simulink model "Set_Speed"  (R2022b)
settings: configuration reference "CommonModelConfiguration" (kept outside this file)
(part 2 of 2)

== stateflow chart Set_Speed/SetSpeed ==
  state CARCONFIG_INVALID
    entry:
    PA_DSF_SetSpeed.Status = E_CommonStatus.NotPresent;
    PA_DSF_SetSpeed.Value = E_DSF_Value.DSF_Off;
    PA_DSF_SetSpeed.SetSpeed = 0;
    PA_DSF_SetSpeed.Offset = 0;
    SET_SetSpdSts = SetSpdSts1.SetSpdSts1_NoReq;
    SET_SetSpdForCrsCtrlFct = 0;
    SET_SetSpdForDispToDrvrVal = 0;
    settings: description=If carconfig isn't fulfilled, which says if there's a driver support function in the car, set the PA:s to the following values.
  state isError = errorCheck [function]
    (default) -> (junction 3420)
    (junction 3420) -> (junction 3421) [order 1] : [(GET_UsrSeldDrvrSpprtFct==DrvrSpprtFct.DrvrSpprtFct_ACC &&...
        | PA_DSF_Adaptive_Cruise_Control_Status==E_CommonStatus.SystemError) ||...
        | (GET_UsrSeldDrvrSpprtFct==DrvrSpprtFct.DrvrSpprtFct_CC &&...
        | PA_DSF_Cruise_Control_Status==E_CommonStatus.SystemError) ||...
        | (GET_UsrSeldDrvrSpprtFct==DrvrSpprtFct.DrvrSpprtFct_SL &&...
        | PA_DSF_Speed_Limiter_Status==E_CommonStatus.SystemError)]
    (junction 3420) -> (junction 3422) [order 2] : {isError = false;}
    (junction 3421) -> (junction 3423) : {isError = true;}
    (junction 3422) -> (junction 3423)
    (junction 3423) -> (junction 3424)
  state SYSTEM_OK
    state isActive = activationCheck [function]
      (default) -> (junction 3433)
      (junction 3433) -> (junction 3434) [order 1] : [(PA_DSF_Speed_Limiter_Status==E_CommonStatus.Available ||...
          | PA_DSF_Cruise_Control_Status==E_CommonStatus.Available ||...
          | PA_DSF_Adaptive_Cruise_Control_Status==E_CommonStatus.Available ||...
          | PA_SpeedControlFunction_Status==E_CommonStatus.Available) &&...
          | (GET_HmiAutnmsStsHmiAutnmsSts~=HmiAutnmsSts1.HmiAutnmsSts1_On ||...
          | cc_param_100~=3)]
      (junction 3433) -> (junction 3435) [order 2] : {isActive = 0;}
      (junction 3434) -> (junction 3436) : {isActive = 1;}
      (junction 3436) -> (junction 3435)
      (junction 3435) -> (junction 3437)
    state NOT_ACTIVE
      entry:
      PA_DSF_SetSpeed.Status = E_CommonStatus.Disabled;
      PA_DSF_SetSpeed.Value = E_DSF_Value.DSF_Off;
      PA_DSF_SetSpeed.SetSpeed = 0;
      PA_DSF_SetSpeed.Offset = 0;
      SET_SetSpdSts = SetSpdSts1.SetSpdSts1_NoReq;
      SET_SetSpdForCrsCtrlFct = 0;
      SET_SetSpdForDispToDrvrVal = 0;
      settings: description=No driver support function is available at the moment
    state ACTIVE
      entry:
      SET_SetSpdSts = SetSpdSts1.SetSpdSts1_NoReq;
      state ACTIVE_A2
        state MAX_AND_MIN_SETSPEED [parallel]
          %Sets the max and min set speed
          %the entry transition can be where ever, the correct value-
          %will be set the next step
          settings: executionOrder=1
          state retVal =MinSpeed(LCFG_SpeedMPH, LCFG_SpeedKPH) [function]
            (default) -> (junction 5350)
            (junction 5350) -> (junction 5351) [order 1] : [GET_SpdUnit==VehSpdIndcdUnit.VehSpdIndcdUnit_Kmph]
            (junction 5350) -> (junction 5352) [order 2] : {retVal=LCFG_SpeedMPH;}
            (junction 5351) -> (junction 5353) : {retVal=LCFG_SpeedKPH;}
            (junction 5353) -> (junction 5352)
            (junction 5352) -> (junction 5354)
            (junction 5354) -> (junction 5355) [order 1] : [retVal>CARCONFIG_MaxSetSpeed(cc_param_43)]
            (junction 5354) -> (junction 5356) [order 2]
            (junction 5355) -> (junction 5357) : {retVal=CARCONFIG_MaxSetSpeed(cc_param_43);}
            (junction 5357) -> (junction 5356)
            (junction 5356) -> (junction 5358)
          state retVal=Max_SetSpeed(LCFG_MPH, LCFG_KMPH) [function]
            (default) -> (junction 5374)
            (junction 5374) -> (junction 5375) [order 1] : [GET_SpdUnit==VehSpdIndcdUnit.VehSpdIndcdUnit_Mph]
            (junction 5374) -> (junction 5376) [order 2]
            (junction 5375) -> (junction 5378)
            (junction 5376) -> (junction 5377) [order 1] : [LCFG_KMPH>CARCONFIG_MaxSetSpeed(cc_param_43)]
            (junction 5378) -> (junction 5377) [order 1] : [LCFG_MPH>CARCONFIG_MaxSetSpeed(cc_param_43)]
            (junction 5376) -> (junction 5379) [order 2] : {retVal=LCFG_KMPH;}
            (junction 5377) -> (junction 5380) : {retVal=CARCONFIG_MaxSetSpeed(cc_param_43);}
            (junction 5378) -> (junction 5381) [order 2] : {retVal=LCFG_MPH;}
            (junction 5380) -> (junction 5379)
            (junction 5381) -> (junction 5380)
            (junction 5379) -> (junction 5382)
          state retval=CareKey(MaxSetSpeed) [function]
            (default) -> (junction 5401)
            (junction 5401) -> (junction 5402) [order 1] : [PA_VS_ReducedMaxSpeed_Status==E_CommonStatus.Available]
            (junction 5402) -> (junction 5403) [order 1] : [(GET_SpdUnit==VehSpdIndcdUnit.VehSpdIndcdUnit_Kmph &&...
                | SetSpeedMin<GET_KeyRstrictdActvSpeedLimit*(36/10)) ||...
                | (GET_SpdUnit==VehSpdIndcdUnit.VehSpdIndcdUnit_Mph &&...
                | SetSpeedMin<GET_KeyRstrictdActvSpeedLimit*(1152/512))]
            (junction 5401) -> (junction 5408) [order 2] : {retval=MaxSetSpeed}
            (junction 5402) -> (junction 5409) [order 2] : {retval=SetSpeedMin}
            (junction 5403) -> (junction 5405)
            (junction 5405) -> (junction 5404) [order 2] : [GET_SpdUnit==VehSpdIndcdUnit.VehSpdIndcdUnit_Kmph &&...
                | MaxSetSpeed>GET_KeyRstrictdActvSpeedLimit*(36/10)]
            (junction 5405) -> (junction 5406) [order 1] : [GET_SpdUnit==VehSpdIndcdUnit.VehSpdIndcdUnit_Mph &&...
                | MaxSetSpeed>GET_KeyRstrictdActvSpeedLimit*(1152/512)]
            (junction 5404) -> (junction 5407) : {retval=GET_KeyRstrictdActvSpeedLimit*(36/10)}
            (junction 5405) -> (junction 5410) [order 3] : {retval=MaxSetSpeed}
            (junction 5406) -> (junction 5411) : {retval=GET_KeyRstrictdActvSpeedLimit*(1152/512)}
            (junction 5407) -> (junction 5409)
            (junction 5410) -> (junction 5407)
            (junction 5411) -> (junction 5410)
            (junction 5409) -> (junction 5408)
            (junction 5408) -> (junction 5412)
          state CC
            entry, during: SetSpeedMin= MinSpeed(LCFG_CC_SetSpeedMinMPH, LCFG_CC_SetSpeedMinKPH);
            SetSpeedMax=CareKey(Max_SetSpeed(LCFG_CC_SetSpeedMaxMPH, LCFG_CC_SetSpeedMaxKPH));
          state SL
            entry, during: SetSpeedMin=MinSpeed(LCFG_SL_SetSpeedMinMPH, LCFG_SL_SetSpeedMinKPH);
            SetSpeedMax =CareKey( CARCONFIG_MaxSetSpeed(cc_param_43));
          state ACC
            entry, during: SetSpeedMin=MinSpeed(LCFG_SetSpeedMinMPH, LCFG_SetSpeedMinKPH);
            SetSpeedMax=CareKey(Max_SetSpeed(LCFG_SetSpeedMaxMPH, LCFG_SetSpeedMaxKPH));
          SYSTEM_OK.ACTIVE.ACTIVE_A2.MAX_AND_MIN_SETSPEED.ACC -> CC [order 1] : [PA_DSF_Cruise_Control_Status==E_CommonStatus.Available]
          CC -> SYSTEM_OK.ACTIVE.ACTIVE_A2.MAX_AND_MIN_SETSPEED.ACC [order 1] : [PA_DSF_Adaptive_Cruise_Control_Status==E_CommonStatus.Available]
          SYSTEM_OK.ACTIVE.ACTIVE_A2.MAX_AND_MIN_SETSPEED.SL -> CC [order 1] : [PA_DSF_Cruise_Control_Status==E_CommonStatus.Available]
          CC -> SYSTEM_OK.ACTIVE.ACTIVE_A2.MAX_AND_MIN_SETSPEED.SL [order 2] : [PA_DSF_Speed_Limiter_Status==E_CommonStatus.Available]
          (default) -> SYSTEM_OK.ACTIVE.ACTIVE_A2.MAX_AND_MIN_SETSPEED.ACC
          SYSTEM_OK.ACTIVE.ACTIVE_A2.MAX_AND_MIN_SETSPEED.SL -> SYSTEM_OK.ACTIVE.ACTIVE_A2.MAX_AND_MIN_SETSPEED.ACC [order 2] : [PA_DSF_Adaptive_Cruise_Control_Status==E_CommonStatus.Available]
          SYSTEM_OK.ACTIVE.ACTIVE_A2.MAX_AND_MIN_SETSPEED.ACC -> SYSTEM_OK.ACTIVE.ACTIVE_A2.MAX_AND_MIN_SETSPEED.SL [order 2] : [PA_DSF_Speed_Limiter_Status==E_CommonStatus.Available]
        state SETSPEED_HANDLING [parallel]
          entry: PA_DSF_SetSpeed.Status=E_CommonStatus.Available;
          PA_DSF_SetSpeed.Value=E_DSF_Value.DSF_Off;
          LCFG_Unit_Check();
          manualUpdate = false;
          during: unitChange();
          settings: executionOrder=2
          state SLA_UPDATE [parallel]
            during: Reset_Offset()
            settings: executionOrder=1
            state SETSPEED_REASON_RESET_COUNTER
            state SETSPEED_REASON_RESET
              entry: SET_SetSpdSts = SetSpdSts1.SetSpdSts1_NoReq;
            (default) -> SETSPEED_REASON_RESET
            SETSPEED_REASON_RESET -> SETSPEED_REASON_RESET_COUNTER : [slaUpdate()]
            SETSPEED_REASON_RESET_COUNTER -> SETSPEED_REASON_RESET [order 1] : [after(250, msec)]
            SETSPEED_REASON_RESET_COUNTER -> SETSPEED_REASON_RESET_COUNTER [order 2] : [slaUpdate()]
          state MANUAL_UPDATE [parallel]
            settings: executionOrder=2
            state OFF
              state STANDBY
                entry: PA_DSF_SetSpeed.Value=E_DSF_Value.DSF_Standby;
                manualUpdate = false;
            state ACTIVE
              entry,during: updateValue()
              state REQ_DISABLED
              state updateValue [function]
                (default) -> (junction 4911)
                (junction 4911) -> (junction 4910) [order 1] : [PA_DSF_Adaptive_Cruise_Control_Value == E_DSF_Value.DSF_StopMode]
                    |
                    | {PA_DSF_SetSpeed.Value = E_DSF_Value.DSF_Standby;}
                (junction 4910) -> (junction 4915)
                (junction 4911) -> (junction 4913) [order 2]
                (junction 4913) -> (junction 4912) [order 1] : [PA_DSF_SL_Warning_Value == E_OffOn.On ||...
                    | GET_AdjSpdLimnSts==AdjSpdLimnSts2.AdjSpdLimnSts2_Ovrd]
                    |
                    | {PA_DSF_SetSpeed.Value = E_DSF_Value.DSF_Overridden;}
                (junction 4912) -> (junction 4914)
                (junction 4913) -> (junction 4916) [order 2] : {PA_DSF_SetSpeed.Value = E_DSF_Value.DSF_Active;}
                (junction 4915) -> (junction 4914)
                (junction 4914) -> (junction 4916)
                (junction 4916) -> (junction 4917)
              state IDLE
                entry:
                manualUpdate = false;
                settings: description=In this state the application is waiting for steering wheel button events
              state SET_CURRENT_SPEED
                entry: PA_DSF_SetSpeed.SetSpeed = setCruiseSpeed(GET_VehSpdIndcdVal);
                SET_SetSpdSts = SetSpdSts1.SetSpdSts1_DrvrReq;
                manualUpdate = true;
              state SPEED_TAP
                entry: SET_SetSpdSts = SetSpdSts1.SetSpdSts1_DrvrReq;
                manualUpdate = true;
                settings: description="In this state the cruise speed is increased/decreased the amount specified by the Local Config parameter \"SetSpeedTap)"
                state retval=getIncrease(reqsetspeed) [function]
                  (default) -> (junction 4959) : {retval = setCruiseSpeed(reqsetspeed+ SetSpeedTap -...
                      | mod(reqsetspeed, SetSpeedTap));}
                state retval=getDecrease(reqsetspeed) [function]
                  (default) -> (junction 4964)
                  (junction 4964) -> (junction 4965) [order 1] : [mod(reqsetspeed, SetSpeedTap) > 0]
                  (junction 4964) -> (junction 4966) [order 2] : {retval = setCruiseSpeed(reqsetspeed - SetSpeedTap);}
                  (junction 4965) -> (junction 4967) : {retval = setCruiseSpeed(reqsetspeed -...
                      | mod(reqsetspeed, SetSpeedTap));}
                  (junction 4967) -> (junction 4966)
                  (junction 4966) -> (junction 4968)
                (default) -> (junction 4932)
                (junction 4932) -> (junction 4931) [order 1] : [INT_SWSInputData.Button == E_SWSButton.BtnL4Req]
                (junction 4931) -> (junction 4933)
                (junction 4932) -> (junction 4934) [order 2]
                (junction 4933) -> (junction 4936) [order 1] : [PA_DSF_Speed_Limit_Adaptation_Data~=0 && PA_DSF_Speed_Limit_Adaptation_Data<254 &&...
                    | PA_DSF_Speed_Limit_Adaptation_Value== E_DSF_Value.DSF_Active]
                (junction 4934) -> (junction 4935) [order 1] : [PA_DSF_Speed_Limit_Adaptation_Data~=0 && PA_DSF_Speed_Limit_Adaptation_Data<254 &&...
                    | PA_DSF_Speed_Limit_Adaptation_Value== E_DSF_Value.DSF_Active]
                (junction 4933) -> (junction 4937) [order 2] : {PA_DSF_SetSpeed.SetSpeed = getDecrease(PA_DSF_SetSpeed.SetSpeed);}
                (junction 4934) -> (junction 4938) [order 2] : {PA_DSF_SetSpeed.SetSpeed =getIncrease(PA_DSF_SetSpeed.SetSpeed);}
                (junction 4935) -> (junction 4939) : {PA_DSF_SetSpeed.Offset = setMaxSlOffset(getIncrease(setCruiseSpeed(SLA_Sign_Value)...
                    | + PA_DSF_SetSpeed.Offset) - setCruiseSpeed(SLA_Sign_Value));
                    | PA_DSF_SetSpeed.SetSpeed = setCruiseSpeed(SLA_Sign_Value)...
                    | + PA_DSF_SetSpeed.Offset;}
                (junction 4936) -> (junction 4940) : {PA_DSF_SetSpeed.Offset = setMaxSlOffset(getDecrease(setCruiseSpeed(SLA_Sign_Value)...
                    | + PA_DSF_SetSpeed.Offset) - setCruiseSpeed(SLA_Sign_Value));
                    | PA_DSF_SetSpeed.SetSpeed = setCruiseSpeed(SLA_Sign_Value) + PA_DSF_SetSpeed.Offset;}
                (junction 4940) -> (junction 4937)
                (junction 4937) -> (junction 4939)
                (junction 4939) -> (junction 4938)
                (junction 4938) -> (junction 4941)
              state SPEED_RAMP
                entry: fineTuningDone = false;
                SET_SetSpdSts = SetSpdSts1.SetSpdSts1_DrvrReq;
                manualUpdate = true;
                state ramp [function]
                  (default) -> (junction 4982)
                  (junction 4982) -> (junction 4983) [order 1] : [INT_SWSInputData.Button == E_SWSButton.BtnL4Req]
                  (junction 4982) -> (junction 4986) [order 2]
                  (junction 4983) -> (junction 4985)
                  (junction 4985) -> (junction 4984) [order 1] : [PA_DSF_Speed_Limit_Adaptation_Data~=0 && PA_DSF_Speed_Limit_Adaptation_Data<254 &&...
                      | (PA_DSF_Speed_Limit_Adaptation_Value== E_DSF_Value.DSF_Active)]
                  (junction 4984) -> (junction 4988) : {PA_DSF_SetSpeed.Offset = setMaxSlOffset(setCruiseSpeed(setCruiseSpeed(SLA_Sign_Value)...
                      | + PA_DSF_SetSpeed.Offset - SetSpeedRamp) - setCruiseSpeed(SLA_Sign_Value));
                      | PA_DSF_SetSpeed.SetSpeed = setCruiseSpeed(SLA_Sign_Value) + PA_DSF_SetSpeed.Offset;}
                  (junction 4985) -> (junction 4989) [order 2] : {PA_DSF_SetSpeed.SetSpeed = setCruiseSpeed(PA_DSF_SetSpeed.SetSpeed - SetSpeedRamp);}
                  (junction 4986) -> (junction 4987) [order 1] : [PA_DSF_Speed_Limit_Adaptation_Data~=0 && PA_DSF_Speed_Limit_Adaptation_Data<254 &&...
                      | PA_DSF_Speed_Limit_Adaptation_Value== E_DSF_Value.DSF_Active]
                  (junction 4987) -> (junction 4991) : {PA_DSF_SetSpeed.Offset = setMaxSlOffset(setCruiseSpeed(setCruiseSpeed(SLA_Sign_Value)...
                      | + PA_DSF_SetSpeed.Offset + SetSpeedRamp) - setCruiseSpeed(SLA_Sign_Value));
                      | PA_DSF_SetSpeed.SetSpeed = setCruiseSpeed(SLA_Sign_Value)...
                      | + PA_DSF_SetSpeed.Offset;}
                  (junction 4986) -> (junction 4990) [order 2] : {PA_DSF_SetSpeed.SetSpeed =setCruiseSpeed(PA_DSF_SetSpeed.SetSpeed+SetSpeedRamp);}
                  (junction 4988) -> (junction 4989)
                  (junction 4989) -> (junction 4991)
                  (junction 4991) -> (junction 4990)
                  (junction 4990) -> (junction 4992)
                state HOLD_SHORT
                  state IDLE
                  state RAMP
                    entry: ramp()
                  (default) -> SYSTEM_OK.ACTIVE.ACTIVE_A2.SETSPEED_HANDLING.MANUAL_UPDATE.ACTIVE.SPEED_RAMP.HOLD_SHORT.RAMP
                  SYSTEM_OK.ACTIVE.ACTIVE_A2.SETSPEED_HANDLING.MANUAL_UPDATE.ACTIVE.SPEED_RAMP.HOLD_SHORT.RAMP -> SYSTEM_OK.ACTIVE.ACTIVE_A2.SETSPEED_HANDLING.MANUAL_UPDATE.ACTIVE.SPEED_RAMP.HOLD_SHORT.IDLE
                  SYSTEM_OK.ACTIVE.ACTIVE_A2.SETSPEED_HANDLING.MANUAL_UPDATE.ACTIVE.SPEED_RAMP.HOLD_SHORT.IDLE -> SYSTEM_OK.ACTIVE.ACTIVE_A2.SETSPEED_HANDLING.MANUAL_UPDATE.ACTIVE.SPEED_RAMP.HOLD_SHORT.RAMP : after(LCFG_AdjustmentShort, sec)
                state HOLD_LONG_ADJUST_SPEED
                  state IDLE
                  state RAMP
                    entry: ramp()
                  (default) -> SYSTEM_OK.ACTIVE.ACTIVE_A2.SETSPEED_HANDLING.MANUAL_UPDATE.ACTIVE.SPEED_RAMP.HOLD_LONG_ADJUST_SPEED.IDLE
                  SYSTEM_OK.ACTIVE.ACTIVE_A2.SETSPEED_HANDLING.MANUAL_UPDATE.ACTIVE.SPEED_RAMP.HOLD_LONG_ADJUST_SPEED.RAMP -> SYSTEM_OK.ACTIVE.ACTIVE_A2.SETSPEED_HANDLING.MANUAL_UPDATE.ACTIVE.SPEED_RAMP.HOLD_LONG_ADJUST_SPEED.IDLE
                  SYSTEM_OK.ACTIVE.ACTIVE_A2.SETSPEED_HANDLING.MANUAL_UPDATE.ACTIVE.SPEED_RAMP.HOLD_LONG_ADJUST_SPEED.IDLE -> SYSTEM_OK.ACTIVE.ACTIVE_A2.SETSPEED_HANDLING.MANUAL_UPDATE.ACTIVE.SPEED_RAMP.HOLD_LONG_ADJUST_SPEED.RAMP : after(LCFG_AdjustmentLong, sec)
                state FINE_TUNING
                  state FINE_TUNING_DONE
                    entry: fineTuningDone = true
                  state No_RELEASE
                  state RAMP
                  (default) -> SYSTEM_OK.ACTIVE.ACTIVE_A2.SETSPEED_HANDLING.MANUAL_UPDATE.ACTIVE.SPEED_RAMP.FINE_TUNING.RAMP
                  SYSTEM_OK.ACTIVE.ACTIVE_A2.SETSPEED_HANDLING.MANUAL_UPDATE.ACTIVE.SPEED_RAMP.FINE_TUNING.RAMP -> SYSTEM_OK.ACTIVE.ACTIVE_A2.SETSPEED_HANDLING.MANUAL_UPDATE.ACTIVE.SPEED_RAMP.FINE_TUNING.No_RELEASE : [INT_SWSInputData.Event~=E_SWSEvent.Release]
                  SYSTEM_OK.ACTIVE.ACTIVE_A2.SETSPEED_HANDLING.MANUAL_UPDATE.ACTIVE.SPEED_RAMP.FINE_TUNING.No_RELEASE -> SYSTEM_OK.ACTIVE.ACTIVE_A2.SETSPEED_HANDLING.MANUAL_UPDATE.ACTIVE.SPEED_RAMP.FINE_TUNING.FINE_TUNING_DONE [order 2] : after(LCFG_FineTuning, sec)
                  (junction 5020) -> SYSTEM_OK.ACTIVE.ACTIVE_A2.SETSPEED_HANDLING.MANUAL_UPDATE.ACTIVE.SPEED_RAMP.FINE_TUNING.RAMP
                  SYSTEM_OK.ACTIVE.ACTIVE_A2.SETSPEED_HANDLING.MANUAL_UPDATE.ACTIVE.SPEED_RAMP.FINE_TUNING.No_RELEASE -> (junction 5021) [order 1] : [INT_SWSInputData.Event==E_SWSEvent.Release]
                  (junction 5021) -> (junction 5020) : {ramp()}
                (default) -> SYSTEM_OK.ACTIVE.ACTIVE_A2.SETSPEED_HANDLING.MANUAL_UPDATE.ACTIVE.SPEED_RAMP.HOLD_SHORT
                SYSTEM_OK.ACTIVE.ACTIVE_A2.SETSPEED_HANDLING.MANUAL_UPDATE.ACTIVE.SPEED_RAMP.HOLD_SHORT -> SYSTEM_OK.ACTIVE.ACTIVE_A2.SETSPEED_HANDLING.MANUAL_UPDATE.ACTIVE.SPEED_RAMP.HOLD_LONG_ADJUST_SPEED [order 1] : [INT_SWSInputData.Event == E_SWSEvent.HoldLong]
                SYSTEM_OK.ACTIVE.ACTIVE_A2.SETSPEED_HANDLING.MANUAL_UPDATE.ACTIVE.SPEED_RAMP.FINE_TUNING -> SYSTEM_OK.ACTIVE.ACTIVE_A2.SETSPEED_HANDLING.MANUAL_UPDATE.ACTIVE.SPEED_RAMP.HOLD_SHORT : [INT_SWSInputData.Event == E_SWSEvent.HoldShort]
                SYSTEM_OK.ACTIVE.ACTIVE_A2.SETSPEED_HANDLING.MANUAL_UPDATE.ACTIVE.SPEED_RAMP.HOLD_SHORT -> SYSTEM_OK.ACTIVE.ACTIVE_A2.SETSPEED_HANDLING.MANUAL_UPDATE.ACTIVE.SPEED_RAMP.FINE_TUNING [order 2] : [INT_SWSInputData.Event == E_SWSEvent.Release]
                SYSTEM_OK.ACTIVE.ACTIVE_A2.SETSPEED_HANDLING.MANUAL_UPDATE.ACTIVE.SPEED_RAMP.HOLD_LONG_ADJUST_SPEED -> SYSTEM_OK.ACTIVE.ACTIVE_A2.SETSPEED_HANDLING.MANUAL_UPDATE.ACTIVE.SPEED_RAMP.FINE_TUNING : [INT_SWSInputData.Event == E_SWSEvent.Release]
              (default) -> SYSTEM_OK.ACTIVE.ACTIVE_A2.SETSPEED_HANDLING.MANUAL_UPDATE.ACTIVE.REQ_DISABLED
              SYSTEM_OK.ACTIVE.ACTIVE_A2.SETSPEED_HANDLING.MANUAL_UPDATE.ACTIVE.IDLE -> SYSTEM_OK.ACTIVE.ACTIVE_A2.SETSPEED_HANDLING.MANUAL_UPDATE.ACTIVE.REQ_DISABLED [order 1] : [GET_AccSts==AccSts1.AccSts1_Stop ||...
                  | GET_AccSts==AccSts1.AccSts1_StopTmp]
              SYSTEM_OK.ACTIVE.ACTIVE_A2.SETSPEED_HANDLING.MANUAL_UPDATE.ACTIVE.REQ_DISABLED -> SYSTEM_OK.ACTIVE.ACTIVE_A2.SETSPEED_HANDLING.MANUAL_UPDATE.ACTIVE.IDLE : [INT_SWSInputData.Event == E_SWSEvent.Idle &&...
                  | GET_AccSts~=AccSts1.AccSts1_Stop &&...
                  | GET_AccSts~=AccSts1.AccSts1_StopTmp]
              SYSTEM_OK.ACTIVE.ACTIVE_A2.SETSPEED_HANDLING.MANUAL_UPDATE.ACTIVE.IDLE -> SYSTEM_OK.ACTIVE.ACTIVE_A2.SETSPEED_HANDLING.MANUAL_UPDATE.ACTIVE.SET_CURRENT_SPEED [order 2] : [(PA_DSF_Cruise_Control_Status==E_CommonStatus.Available ||...
                  | PA_DSF_Adaptive_Cruise_Control_Status==E_CommonStatus.Available) &&...
                  | GET_CrsCtrlOvrdn==OnOff1.OnOff1_On &&...
                  | INT_SWSInputData.Button == E_SWSButton.BtnL5Req &&...
                  | INT_SWSInputData.Event == E_SWSEvent.Push &&...
                  | GET_VehSpdIndcdVal>=PA_DSF_SetSpeed.SetSpeed]
              SYSTEM_OK.ACTIVE.ACTIVE_A2.SETSPEED_HANDLING.MANUAL_UPDATE.ACTIVE.SET_CURRENT_SPEED -> SYSTEM_OK.ACTIVE.ACTIVE_A2.SETSPEED_HANDLING.MANUAL_UPDATE.ACTIVE.IDLE : [INT_SWSInputData.Event == E_SWSEvent.Idle]
              SYSTEM_OK.ACTIVE.ACTIVE_A2.SETSPEED_HANDLING.MANUAL_UPDATE.ACTIVE.IDLE -> SYSTEM_OK.ACTIVE.ACTIVE_A2.SETSPEED_HANDLING.MANUAL_UPDATE.ACTIVE.SPEED_TAP [order 3] : [INT_SWSInputData.Event == E_SWSEvent.Release &&...
                  | (INT_SWSInputData.Button == E_SWSButton.BtnL4Req ||...
                  | INT_SWSInputData.Button == E_SWSButton.BtnL5Req)]
                settings: description=If the up or down button, from the left buttons group, is released.
              SYSTEM_OK.ACTIVE.ACTIVE_A2.SETSPEED_HANDLING.MANUAL_UPDATE.ACTIVE.SPEED_TAP -> SYSTEM_OK.ACTIVE.ACTIVE_A2.SETSPEED_HANDLING.MANUAL_UPDATE.ACTIVE.IDLE : [INT_SWSInputData.Event == E_SWSEvent.Idle]
              SYSTEM_OK.ACTIVE.ACTIVE_A2.SETSPEED_HANDLING.MANUAL_UPDATE.ACTIVE.IDLE -> SYSTEM_OK.ACTIVE.ACTIVE_A2.SETSPEED_HANDLING.MANUAL_UPDATE.ACTIVE.SPEED_RAMP [order 4] : [INT_SWSInputData.Event == E_SWSEvent.HoldShort &&...
                  | (INT_SWSInputData.Button == E_SWSButton.BtnL4Req ||...
                  | INT_SWSInputData.Button == E_SWSButton.BtnL5Req)]
              SYSTEM_OK.ACTIVE.ACTIVE_A2.SETSPEED_HANDLING.MANUAL_UPDATE.ACTIVE.SPEED_RAMP -> SYSTEM_OK.ACTIVE.ACTIVE_A2.SETSPEED_HANDLING.MANUAL_UPDATE.ACTIVE.IDLE : [INT_SWSInputData.Event == E_SWSEvent.Idle && fineTuningDone]
            (default) -> SYSTEM_OK.ACTIVE.ACTIVE_A2.SETSPEED_HANDLING.MANUAL_UPDATE.OFF
            SYSTEM_OK.ACTIVE.ACTIVE_A2.SETSPEED_HANDLING.MANUAL_UPDATE.ACTIVE -> STANDBY : [PA_DSF_Cruise_Control_Value==E_DSF_Value.DSF_Standby ||...
                | PA_DSF_Speed_Limiter_Value==E_DSF_Value.DSF_Standby ||...
                | PA_DSF_Adaptive_Cruise_Control_Value==E_DSF_Value.DSF_Standby]
            SYSTEM_OK.ACTIVE.ACTIVE_A2.SETSPEED_HANDLING.MANUAL_UPDATE.OFF -> SYSTEM_OK.ACTIVE.ACTIVE_A2.SETSPEED_HANDLING.MANUAL_UPDATE.ACTIVE [order 1] : [hasChangedTo(INT_CC_Event, E_DSF_Event.Activation) ||...
                | (PA_DSF_Cruise_Control_Value==E_DSF_Value.DSF_Active &&...
                | INT_CC_Event ==E_DSF_Event.NoReq) ||...
                | hasChangedTo(INT_SL_Event, E_DSF_Event.Activation) ||...
                | (PA_DSF_Speed_Limiter_Value==E_DSF_Value.DSF_Active &&...
                | INT_SL_Event ==E_DSF_Event.NoReq) ||...
                | hasChangedTo(INT_ACC_Event, E_DSF_Event.Activation) ||...
                | ((PA_DSF_Adaptive_Cruise_Control_Value==E_DSF_Value.DSF_Active ||...
                | PA_DSF_Adaptive_Cruise_Control_Value==E_DSF_Value.DSF_StopMode) &&...
                | INT_ACC_Event == E_DSF_Event.NoReq)]
                | {setDsfActivation()}
            SYSTEM_OK.ACTIVE.ACTIVE_A2.SETSPEED_HANDLING.MANUAL_UPDATE.OFF -> SYSTEM_OK.ACTIVE.ACTIVE_A2.SETSPEED_HANDLING.MANUAL_UPDATE.ACTIVE [order 2] : [hasChangedTo(INT_CC_Event, E_DSF_Event.Resume) ||...
                | hasChangedTo(INT_SL_Event, E_DSF_Event.Resume) ||...
                | hasChangedTo(INT_ACC_Event, E_DSF_Event.Resume)]
          state SLA_Speed_Change [function]
            state slaSetSpeedChange [function]
              (default) -> (junction 5076)
              (junction 5076) -> (junction 5077) [order 1] : [GET_SetSpdSelnForAutDrv==SetSpdSelnForAutDrv1.SetSpdSelnForAutDrv1_AdjSetSpdToCmngSpdLim]
              (junction 5076) -> (junction 5078) [order 2] : {SET_SetSpdSts = SetSpdSts1.SetSpdSts1_Lvl1;}
              (junction 5077) -> (junction 5079) : {SET_SetSpdSts = SetSpdSts1.SetSpdSts1_Lvl2;}
              (junction 5079) -> (junction 5078)
              (junction 5078) -> (junction 5080)
            (default) -> (junction 5040)
            (junction 5040) -> (junction 5039) [order 2]
            (junction 5040) -> (junction 5041) [order 1] : [PA_DSF_Adaptive_Cruise_Control_Status==E_CommonStatus.Available]
            (junction 5039) -> (junction 5043)
            (junction 5041) -> (junction 5044)
            (junction 5043) -> (junction 5042) [order 1] : [LCFG_SL_OffsetReset==false]
            (junction 5044) -> (junction 5045) [order 1] : [PA_DSF_Speed_Limit_Adaptation_Value~=E_DSF_Value.DSF_Standby]
            (junction 5043) -> (junction 5049) [order 2] : {PA_DSF_SetSpeed.SetSpeed=setCruiseSpeed(SLA_Sign_Value);
                | PA_DSF_SetSpeed.Offset=0;
                | SET_SetSpdSts = SetSpdSts1.SetSpdSts1_Lvl1;}
            (junction 5044) -> (junction 5051) [order 2] : {PA_DSF_SetSpeed.SetSpeed = setCruiseSpeed(GET_VehSpdIndcdVal - PA_DSF_SetSpeed.Offset);}
            (junction 5045) -> (junction 5046)
            (junction 5042) -> (junction 5048) : {PA_DSF_SetSpeed.Offset = setMaxSlOffset(setCruiseSpeed(setCruiseSpeed(SLA_Sign_Value)...
                | + PA_DSF_SetSpeed.Offset) - setCruiseSpeed(SLA_Sign_Value));
                | PA_DSF_SetSpeed.SetSpeed = setCruiseSpeed(SLA_Sign_Value)...
                | + PA_DSF_SetSpeed.Offset;
                | SET_SetSpdSts = SetSpdSts1.SetSpdSts1_Lvl1;}
            (junction 5046) -> (junction 5047) [order 1] : [PA_DSF_Speed_Limit_Adaptation_Data==254]
            (junction 5046) -> (junction 5052) [order 2] : {PA_DSF_SetSpeed.Offset = setCruiseSpeed(setCruiseSpeed(SLA_Sign_Value)...
                | + PA_DSF_SetSpeed.Offset) - setCruiseSpeed(SLA_Sign_Value);
                | PA_DSF_SetSpeed.SetSpeed = setCruiseSpeed(SLA_Sign_Value)...
                | + PA_DSF_SetSpeed.Offset;
                | slaSetSpeedChange()}
            (junction 5047) -> (junction 5053) : {PA_DSF_SetSpeed.Offset=0;
                | slaSetSpeedChange()}
            (junction 5048) -> (junction 5049)
            (junction 5049) -> (junction 5050)
            (junction 5051) -> (junction 5050)
            (junction 5052) -> (junction 5051)
            (junction 5053) -> (junction 5052)
            (junction 5050) -> (junction 5054)
          state retVal=slaUpdate [function]
            (default) -> (junction 5090)
            (junction 5090) -> (junction 5089) [order 1] : [hasChangedTo(PA_DSF_Speed_Limit_Adaptation_Value, E_DSF_Value.DSF_Standby)]
            (junction 5089) -> (junction 5098) : {retVal=false;
                | SLA_Speed_Change()}
            (junction 5090) -> (junction 5091) [order 2]
            (junction 5091) -> (junction 5092) [order 1] : [PA_DSF_Speed_Limit_Adaptation_Data~=0 &&...
                | PA_DSF_Speed_Limit_Adaptation_Data~=255]
            (junction 5091) -> (junction 5093) [order 2]
            (junction 5092) -> (junction 5094)
            (junction 5094) -> (junction 5095) [order 1] : [(PA_DSF_SetSpeed.SetSpeed~=0 &&...
                | hasChanged(PA_DSF_Speed_Limit_Adaptation_Data) &&...
                | (PA_DSF_Speed_Limit_Adaptation_Value==E_DSF_Value.DSF_Active ||...
                | PA_DSF_Speed_Limit_Adaptation_Value==E_DSF_Value.DSF_Selected)) ||...
                | hasChangedTo(PA_DSF_Speed_Limit_Adaptation_Value, E_DSF_Value.DSF_Active)]
            (junction 5094) -> (junction 5093) [order 2]
            (junction 5093) -> (junction 5096) : {retVal=false;}
            (junction 5095) -> (junction 5097) : {SLA_SpeedValue()
                | SLA_Speed_Change()
                | retVal=true}
            (junction 5097) -> (junction 5096)
            (junction 5098) -> (junction 5097)
            (junction 5096) -> (junction 5099)
            (junction 5099) -> (junction 5100) [order 1] : [manualUpdate==true]
            (junction 5099) -> (junction 5101) [order 2]
            (junction 5100) -> (junction 5102) : {retVal = true;}
            (junction 5102) -> (junction 5101)
            (junction 5101) -> (junction 5103)
          state SLA_SpeedValue [function]
            (default) -> (junction 5124) : {SLA_Sign_Value=PA_DSF_Speed_Limit_Adaptation_Data}
            (junction 5124) -> (junction 5125) [order 1] : [(GET_SpdLimUnit==SpdUnit1.SpdUnit1_KiloMtrPerHr &&...
                | GET_SpdUnit==VehSpdIndcdUnit.VehSpdIndcdUnit_Mph) ||...
                | (GET_SpdLimUnit==SpdUnit1.SpdUnit1_MilePerHr &&...
                | GET_SpdUnit==VehSpdIndcdUnit.VehSpdIndcdUnit_Kmph)]
            (junction 5124) -> (junction 5128) [order 2]
            (junction 5125) -> (junction 5126)
            (junction 5126) -> (junction 5127) [order 1] : [GET_SpdLimUnit==SpdUnit1.SpdUnit1_KiloMtrPerHr]
            (junction 5126) -> (junction 5129) [order 2] : {SLA_Sign_Value=103/64*SLA_Sign_Value;}
            (junction 5127) -> (junction 5130) : {SLA_Sign_Value=64/103*SLA_Sign_Value;}
            (junction 5129) -> (junction 5128) : {SLA_Sign_Value= floor(SLA_Sign_Value);}
                | %Round down to nearest integer
            (junction 5130) -> (junction 5129)
            (junction 5128) -> (junction 5131)
          state Reset_Offset [function]
            (default) -> (junction 5143)
            (junction 5143) -> (junction 5144) [order 1] : [PA_DSF_Speed_Limit_Adaptation_Value~= E_DSF_Value.DSF_Active &&...
                | PA_DSF_Speed_Limit_Adaptation_Value~= E_DSF_Value.DSF_Selected &&...
                | PA_DSF_Speed_Limit_Adaptation_Value~= E_DSF_Value.DSF_Standby]
            (junction 5144) -> (junction 5146) : {PA_DSF_SetSpeed.SetSpeed = PA_DSF_SetSpeed.SetSpeed...
                | - PA_DSF_SetSpeed.Offset;
                | PA_DSF_SetSpeed.Offset = 0;}
            (junction 5143) -> (junction 5145) [order 2]
            (junction 5146) -> (junction 5145)
            (junction 5145) -> (junction 5147)
          state retval=setMaxSlOffset(reqoffset) [function]
            state offset_max=LCFG_Offset [function]
              (default) -> (junction 5197)
              (junction 5197) -> (junction 5196) [order 1] : [GET_SpdUnit==VehSpdIndcdUnit.VehSpdIndcdUnit_Mph]
              (junction 5196) -> (junction 5198) : {offset_max=LCFG_SL_MaxOffsetMPH}
              (junction 5197) -> (junction 5199) [order 2] : {offset_max=LCFG_SL_MaxOffsetKPH}
              (junction 5198) -> (junction 5199)
              (junction 5199) -> (junction 5200)
            (default) -> (junction 5176)
            (junction 5176) -> (junction 5177) [order 1] : [PA_DSF_Speed_Limiter_Status==E_CommonStatus.Available &&...
                | abs(reqoffset)>LCFG_Offset()]
                | %absolute value of reqoffset is greater than LCFG_Offset
            (junction 5176) -> (junction 5180) [order 2] : {retval =reqoffset;}
            (junction 5177) -> (junction 5178)
            (junction 5178) -> (junction 5179) [order 1] : [(reqoffset)>0]
            (junction 5178) -> (junction 5181) [order 2] : {retval=-1*LCFG_Offset();}
            (junction 5179) -> (junction 5182) : {retval=LCFG_Offset();}
            (junction 5181) -> (junction 5180)
            (junction 5182) -> (junction 5181)
            (junction 5180) -> (junction 5183)
          state setDsfActivation [function]
            (default) -> (junction 5155)
            (junction 5155) -> (junction 5156) [order 1] : [SLA_Sign_Value~=0 && SLA_Sign_Value~=255 && (PA_DSF_Speed_Limit_Adaptation_Value== E_DSF_Value.DSF_Active ||...
                |  PA_DSF_Speed_Limit_Adaptation_Value== E_DSF_Value.DSF_Selected)]
            (junction 5155) -> (junction 5157) [order 2]
            (junction 5156) -> (junction 5161) : {PA_DSF_SetSpeed.SetSpeed = setCruiseSpeed(SLA_Sign_Value);
                | PA_DSF_SetSpeed.Offset=0;}
            (junction 5157) -> (junction 5158) [order 1] : [PA_DSF_Adaptive_Cruise_Control_Value==E_DSF_Value.DSF_StopMode]
            (junction 5157) -> (junction 5159) [order 2] : {PA_DSF_SetSpeed.SetSpeed = setCruiseSpeed(GET_VehSpdIndcdVal);}
            (junction 5158) -> (junction 5160) : {PA_DSF_SetSpeed.SetSpeed = setCruiseSpeed(SetSpeedMin);}
            (junction 5160) -> (junction 5159)
            (junction 5161) -> (junction 5160)
            (junction 5159) -> (junction 5162)
          state retval = setCruiseSpeed(val) [function]
            (default) -> (junction 5210)
            (junction 5210) -> (junction 5211)
            (junction 5211) -> (junction 5212) [order 1] : [val < SetSpeedMin]
            (junction 5212) -> (junction 5217) : {retval=SetSpeedMin;}
            (junction 5211) -> (junction 5213) [order 2]
            (junction 5213) -> (junction 5214) [order 1] : [val >SetSpeedMax]
            (junction 5213) -> (junction 5216) [order 2] : {retval=val;}
            (junction 5214) -> (junction 5215) : {retval=SetSpeedMax;}
            (junction 5217) -> (junction 5215)
            (junction 5215) -> (junction 5216)
            (junction 5216) -> (junction 5218)
          state LCFG_Unit_Check [function]
            (default) -> (junction 5231)
            (junction 5231) -> (junction 5232) [order 1] : [GET_SpdUnit==VehSpdIndcdUnit.VehSpdIndcdUnit_Mph]
            (junction 5231) -> (junction 5233) [order 2] : {SetSpeedTap=LCFG_SetSpeedTapKPH;
                | SetSpeedRamp=LCFG_SetSpeedRampKPH;
                | SetSpeedTap2=LCFG_SetSpeedTap2KPH;}
            (junction 5232) -> (junction 5234) : {SetSpeedTap=LCFG_SetSpeedTapMPH;
                | SetSpeedRamp=LCFG_SetSpeedRampMPH;
                | SetSpeedTap2=LCFG_SetSpeedTap2MPH;}
            (junction 5234) -> (junction 5233)
            (junction 5233) -> (junction 5235)
          state unitChange [function]
            (default) -> (junction 5243)
            (junction 5243) -> (junction 5244) [order 1] : [hasChanged(GET_SpdUnit)]
            (junction 5243) -> (junction 5247) [order 2]
            (junction 5244) -> (junction 5245) : {LCFG_Unit_Check();}
            (junction 5245) -> (junction 5246) [order 1] : [GET_SpdUnit==VehSpdIndcdUnit.VehSpdIndcdUnit_Mph]
            (junction 5245) -> (junction 5248) [order 2] : %Convert from MPH to KMPH while making sure we are within
                | % the allowed ranges
                | {PA_DSF_SetSpeed.SetSpeed = setCruiseSpeed(floor(103/64*PA_DSF_SetSpeed.SetSpeed));
                | PA_DSF_SetSpeed.Offset = setMaxSlOffset(floor(103/64*PA_DSF_SetSpeed.Offset));}
            (junction 5246) -> (junction 5249) : %Convert from KMPH to MPH while making sure we are within
                | % the allowed ranges
                | {PA_DSF_SetSpeed.SetSpeed = setCruiseSpeed(floor(64/103*PA_DSF_SetSpeed.SetSpeed));
                | PA_DSF_SetSpeed.Offset = setMaxSlOffset(floor(64/103*PA_DSF_SetSpeed.Offset));}
            (junction 5248) -> (junction 5247)
            (junction 5249) -> (junction 5248)
            (junction 5247) -> (junction 5250)
        state SETSPEED_OUTPUT [parallel]
          entry, during:
          SET_SetSpdForCrsCtrlFct=TrueVehicleSpeed(SetSpeedValue(PA_DSF_SetSpeed.SetSpeed, PA_SpeedControlFunction_Data, PA_SpeedControlFunction_Value));
          SET_SetSpdForDispToDrvrVal=PA_DSF_SetSpeed.SetSpeed;
          settings: executionOrder=3
          state ReqSpeed=SetSpeedValue(SetSpeed, SpeedControlData, SpeedControlValue) [function]
            (default) -> (junction 5267)
            (junction 5267) -> (junction 5268) [order 1] : [SpeedControlValue == E_OffOn.On]
            (junction 5267) -> (junction 5269) [order 2] : {ReqSpeed=SetSpeed;}
            (junction 5268) -> (junction 5270) : {ReqSpeed=SpeedControlData;}
            (junction 5270) -> (junction 5269)
            (junction 5269) -> (junction 5271)
          state ReqSpeed=TrueVehicleSpeed(SetSpeed) [function]
            state ConvertedSpeed = RevertConvertedSetSpeed(ConfigMid, ConfigTop, Speed, BreakpointMid, BreakpointTop) [function]
              (default) -> (junction 5306)
              (junction 5306) -> (junction 5307) [order 1] : [Speed==0]
              (junction 5307) -> (junction 5312) : {ConvertedSpeed=0;}
              (junction 5306) -> (junction 5308) [order 2]
              (junction 5308) -> (junction 5309) [order 1] : [Speed<=BreakpointMid]
              (junction 5308) -> (junction 5310) [order 2] : {ConvertedSpeed=Speed-(Speed-BreakpointMid)*(ConfigTop-ConfigMid)/(BreakpointTop-BreakpointMid)-ConfigMid;}
              (junction 5309) -> (junction 5311) : {ConvertedSpeed=Speed-(Speed*ConfigMid/BreakpointMid);}
              (junction 5311) -> (junction 5310)
              (junction 5312) -> (junction 5311)
              (junction 5310) -> (junction 5313)
            state OutPutSpeed =ConvertToMeterPerSecond (SpeedToConvert) [function]
              (default) -> (junction 5327)
              (junction 5327) -> (junction 5328) [order 1] : [GET_SpdUnit==VehSpdIndcdUnit.VehSpdIndcdUnit_Mph]
              (junction 5327) -> (junction 5329) [order 2] : {OutPutSpeed=SpeedToConvert*10/36;}
              (junction 5328) -> (junction 5330) : {OutPutSpeed=SpeedToConvert*515/1152;}
              (junction 5330) -> (junction 5329)
              (junction 5329) -> (junction 5331)
            (default) -> (junction 5282)
            (junction 5282) -> (junction 5281) [order 1] : [cc_param_160==1 || cc_param_160==3 || cc_param_160==5]
            (junction 5281) -> (junction 5287) : {ReqSpeed=ConvertToMeterPerSecond(SetSpeed);}
            (junction 5282) -> (junction 5283) [order 2]
            (junction 5283) -> (junction 5284) [order 1] : [GET_SpdUnit==VehSpdIndcdUnit.VehSpdIndcdUnit_Kmph]
            (junction 5283) -> (junction 5285) [order 2] : %Convert set speed to kph, remove offset and convert to m/s
                | {ReqSpeed = RevertConvertedSetSpeed(LCFG_AddedVehSpdMidOffset,...
                |  LCFG_AddedVehSpdTopOffset, SetSpeed*(103/64),...
                |  LCFG_AddedVehSpdMidOffset + LCFG_ActualVehSpdMid, ...
                |  LCFG_AddedVehSpdTopOffset + LCFG_ActualVehSpdTop)*10/36;}
            (junction 5284) -> (junction 5286) : %Remove offset and convert to m/s
                | {ReqSpeed = RevertConvertedSetSpeed(LCFG_AddedVehSpdMidOffset,...
                |  LCFG_AddedVehSpdTopOffset, SetSpeed,...
                |  LCFG_AddedVehSpdMidOffset + LCFG_ActualVehSpdMid,...
                |  LCFG_AddedVehSpdTopOffset + LCFG_ActualVehSpdTop)*10/36;}
            (junction 5286) -> (junction 5285)
            (junction 5287) -> (junction 5286)
            (junction 5285) -> (junction 5288)
      state ACTIVE_A3
        entry:
        PA_DSF_SetSpeed.Status = E_CommonStatus.Disabled;
        PA_DSF_SetSpeed.Value = E_DSF_Value.DSF_Off;
        PA_DSF_SetSpeed.SetSpeed = 0;
        PA_DSF_SetSpeed.Offset = 0;
        SET_SetSpdSts = SetSpdSts1.SetSpdSts1_NoReq;
        SET_SetSpdForCrsCtrlFct = 0;
        SET_SetSpdForDispToDrvrVal = 0;
        state MAX_AND_MIN_SETSPEED [parallel]
          %Sets the max and min set speed,
          %the entry transition can be wherever,
          %the correct value will be set the next step
          settings: executionOrder=1
          state retVal = Min_SetSpeed(MinSpeedMPH, MinSpeedKPH) [function]
            (default) -> (junction 4424)
            (junction 4424) -> (junction 4425) [order 1] : [GET_SpdUnit==VehSpdIndcdUnit.VehSpdIndcdUnit_Kmph]
            (junction 4424) -> (junction 4426) [order 2] : {retVal = MinSpeedMPH;}
            (junction 4425) -> (junction 4427) : {retVal = MinSpeedKPH;}
            (junction 4427) -> (junction 4426)
            (junction 4426) -> (junction 4428)
            (junction 4428) -> (junction 4429) [order 1] : [retVal>CARCONFIG_MaxSetSpeed(cc_param_43)]
            (junction 4428) -> (junction 4430) [order 2]
            (junction 4429) -> (junction 4431) : {retVal = CARCONFIG_MaxSetSpeed(cc_param_43);}
            (junction 4431) -> (junction 4430)
            (junction 4430) -> (junction 4432)
          state retVal = Max_SetSpeed(MaxSpeedMPH, MaxSpeedKPH) [function]
            (default) -> (junction 4451)
            (junction 4451) -> (junction 4452) [order 1] : [GET_SpdUnit==VehSpdIndcdUnit.VehSpdIndcdUnit_Mph]
            (junction 4451) -> (junction 4453) [order 2]
            (junction 4452) -> (junction 4455)
            (junction 4453) -> (junction 4454) [order 1] : [MaxSpeedKPH>CARCONFIG_MaxSetSpeed(cc_param_43)]
            (junction 4455) -> (junction 4454) [order 1] : [MaxSpeedMPH>CARCONFIG_MaxSetSpeed(cc_param_43)]
            (junction 4453) -> (junction 4456) [order 2] : {retVal = MaxSpeedKPH;}
            (junction 4454) -> (junction 4457) : {retVal = CARCONFIG_MaxSetSpeed(cc_param_43);}
            (junction 4455) -> (junction 4458) [order 2] : {retVal = MaxSpeedMPH;}
            (junction 4457) -> (junction 4456)
            (junction 4458) -> (junction 4457)
            (junction 4456) -> (junction 4459)
          state retval = CareKey(MaxSetSpeed) [function]
            (default) -> (junction 4475)
            (junction 4475) -> (junction 4476) [order 1] : [PA_VS_ReducedMaxSpeed_Status==...
                | E_CommonStatus.Available]
            (junction 4476) -> (junction 4477) [order 1] : [(GET_SpdUnit==VehSpdIndcdUnit.VehSpdIndcdUnit_Kmph &&...
                | SetSpeedMin<GET_KeyRstrictdActvSpeedLimit*(36/10)) ||...
                | (GET_SpdUnit==VehSpdIndcdUnit.VehSpdIndcdUnit_Mph &&...
                | SetSpeedMin<GET_KeyRstrictdActvSpeedLimit*(1152/512))]
            (junction 4475) -> (junction 4482) [order 2] : {retval = MaxSetSpeed;}
            (junction 4476) -> (junction 4483) [order 2] : {retval = SetSpeedMin;}
            (junction 4477) -> (junction 4479)
            (junction 4479) -> (junction 4478) [order 2] : [GET_SpdUnit==VehSpdIndcdUnit.VehSpdIndcdUnit_Kmph &&...
                | MaxSetSpeed>GET_KeyRstrictdActvSpeedLimit*(36/10)]
            (junction 4479) -> (junction 4480) [order 1] : [GET_SpdUnit==VehSpdIndcdUnit.VehSpdIndcdUnit_Mph &&...
                | MaxSetSpeed>GET_KeyRstrictdActvSpeedLimit*(1152/512)]
            (junction 4478) -> (junction 4481) : {retval = GET_KeyRstrictdActvSpeedLimit*(36/10);}
            (junction 4479) -> (junction 4484) [order 3] : {retval = MaxSetSpeed;}
            (junction 4480) -> (junction 4485) : {retval = GET_KeyRstrictdActvSpeedLimit*(1152/512);}
            (junction 4483) -> (junction 4482)
            (junction 4481) -> (junction 4483)
            (junction 4484) -> (junction 4481)
            (junction 4485) -> (junction 4484)
            (junction 4482) -> (junction 4486)
          state ACC
            entry, during:
            SetSpeedMin =...
            Min_SetSpeed(LCFG_SetSpeedMinMPH_A3, LCFG_SetSpeedMinKPH_A3);
            SetSpeedMax =...
            CareKey(Max_SetSpeed(LCFG_SetSpeedMaxMPH, LCFG_SetSpeedMaxKPH));
          state SL
            entry, during:
            SetSpeedMin =...
            Min_SetSpeed(LCFG_SetSpeedMinMPH_A3, LCFG_SetSpeedMinKPH_A3);
            SetSpeedMax =...
            CareKey(CARCONFIG_MaxSetSpeed(cc_param_43));
          (default) -> SYSTEM_OK.ACTIVE.ACTIVE_A3.MAX_AND_MIN_SETSPEED.ACC
          SYSTEM_OK.ACTIVE.ACTIVE_A3.MAX_AND_MIN_SETSPEED.SL -> SYSTEM_OK.ACTIVE.ACTIVE_A3.MAX_AND_MIN_SETSPEED.ACC : %ACC selected
              | [PA_DSF_Adaptive_Cruise_Control_Status==E_CommonStatus.Available]
          SYSTEM_OK.ACTIVE.ACTIVE_A3.MAX_AND_MIN_SETSPEED.ACC -> SYSTEM_OK.ACTIVE.ACTIVE_A3.MAX_AND_MIN_SETSPEED.SL : %SL selected
              | [PA_DSF_Speed_Limiter_Status==E_CommonStatus.Available]
        state SETSPEED_HANDLING [parallel]
          entry:
          PA_DSF_SetSpeed.Status = E_CommonStatus.Available;
          PA_DSF_SetSpeed.Value = E_DSF_Value.DSF_Off;
          LCFG_Unit_Check();
          during:
          unitChange();
          settings: executionOrder=2
          state MANUAL_UPDATE [parallel]
            settings: executionOrder=1
            state OFF
              entry:
              PA_DSF_SetSpeed.Value =...
              E_DSF_Value.DSF_Standby;
            state ACTIVE
              entry,during: updateValue()
              state REQ_DISABLED
              state updateValue [function]
                (default) -> (junction 4526)
                (junction 4526) -> (junction 4527) [order 1] : [PA_DSF_Adaptive_Cruise_Control_Value==E_DSF_Value.DSF_StopMode]
                    | {PA_DSF_SetSpeed.Value = E_DSF_Value.DSF_Standby;}
                (junction 4526) -> (junction 4528) [order 2]
                (junction 4527) -> (junction 4531)
                (junction 4528) -> (junction 4529) [order 1] : [GET_CrsCtrlOvrdn==OnOff1.OnOff1_On ||...
                    | PA_DSF_SL_Warning_Value==E_OffOn.On ||...
                    | GET_AdjSpdLimnSts==AdjSpdLimnSts2.AdjSpdLimnSts2_Ovrd]
                    | {PA_DSF_SetSpeed.Value = E_DSF_Value.DSF_Overridden;}
                (junction 4529) -> (junction 4530)
                (junction 4528) -> (junction 4532) [order 2] : {PA_DSF_SetSpeed.Value = E_DSF_Value.DSF_Active;}
                (junction 4531) -> (junction 4530)
                (junction 4530) -> (junction 4532)
                (junction 4532) -> (junction 4533)
              state retval = validSLA [function]
                (default) -> (junction 4546) : {retval = PA_DSF_Speed_Limit_Adaptation_Data~=0 &&...
                    | PA_DSF_Speed_Limit_Adaptation_Data<254 &&...
                    | (PA_DSF_Speed_Limit_Adaptation_Value==E_DSF_Value.DSF_Active ||...
                    | PA_DSF_Speed_Limit_Adaptation_Value==E_DSF_Value.DSF_Standby);}
              state offset_max = limitOffset [function]
                (default) -> (junction 4550)
                (junction 4550) -> (junction 4551) [order 1] : [GET_SpdUnit==VehSpdIndcdUnit.VehSpdIndcdUnit_Mph]
                (junction 4550) -> (junction 4552) [order 2] : {offset_max = LCFG_SL_MaxOffsetKPH;}
                (junction 4551) -> (junction 4553) : {offset_max = LCFG_SL_MaxOffsetMPH;}
                (junction 4553) -> (junction 4552)
                (junction 4552) -> (junction 4554)
              state IDLE
                settings: description=In this state the application is waiting for steering wheel button events
              state SET_CURRENT_SPEED
                entry:
                PA_DSF_SetSpeed.SetSpeed = limitCruiseSpeed(GET_VehSpdIndcdVal);
                SET_SetSpdForDispToDrvrVal = PA_DSF_SetSpeed.SetSpeed;
                SetSpeedControlOutput(PA_DSF_SetSpeed.SetSpeed)
              state SPEED_TAP
                settings: description="In this state the cruise speed is increased/decreased the amount specified by the Local Config parameter \"SetSpeedTap)"
                state retval = getIncrease(reqsetspeed) [function]
                  (default) -> (junction 4592) : {retval = limitCruiseSpeed(reqsetspeed + SetSpeedTap -...
                      | mod(reqsetspeed, SetSpeedTap));}
                state retval = getDecrease(reqsetspeed) [function]
                  (default) -> (junction 4597)
                  (junction 4597) -> (junction 4598) [order 1] : [mod(reqsetspeed, SetSpeedTap) > 0]
                  (junction 4597) -> (junction 4599) [order 2] : {retval = limitCruiseSpeed(reqsetspeed - SetSpeedTap);}
                  (junction 4598) -> (junction 4600) : {retval = limitCruiseSpeed(reqsetspeed -...
                      | mod(reqsetspeed, SetSpeedTap));}
                  (junction 4600) -> (junction 4599)
                  (junction 4599) -> (junction 4601)
                (default) -> (junction 4564)
                (junction 4564) -> (junction 4565) [order 1] : %Set speed decrease (down button)
                    | [INT_SWSInputData.Button == E_SWSButton.BtnL4Req]
                (junction 4564) -> (junction 4566) [order 2] : %Set speed increase
                    | {PA_DSF_SetSpeed.SetSpeed = getIncrease(PA_DSF_SetSpeed.SetSpeed);}
                (junction 4565) -> (junction 4568) : %Set speed decrease
                    | {PA_DSF_SetSpeed.SetSpeed = getDecrease(PA_DSF_SetSpeed.SetSpeed);}
                (junction 4566) -> (junction 4567) [order 1] : %SLA valid, SL active and max offset exceeded
                    | [validSLA && PA_DSF_Speed_Limiter_Status==E_CommonStatus.Available &&...
                    | PA_DSF_SetSpeed.SetSpeed - limitCruiseSpeed(SLA_Sign_Value) > limitOffset]
                (junction 4568) -> (junction 4569) [order 1] : %SLA valid, SL active and max offset exceeded
                    | [validSLA && PA_DSF_Speed_Limiter_Status==E_CommonStatus.Available &&...
                    | PA_DSF_SetSpeed.SetSpeed - limitCruiseSpeed(SLA_Sign_Value) < -limitOffset]
                (junction 4566) -> (junction 4570) [order 2]
                (junction 4568) -> (junction 4572) [order 2]
                (junction 4567) -> (junction 4571) : %Limit to max offset from current speed limit
                    | {PA_DSF_SetSpeed.SetSpeed =...
                    | limitCruiseSpeed(SLA_Sign_Value) + limitOffset;}
                (junction 4569) -> (junction 4573) : %Limit to max offset from current speed limit
                    | {PA_DSF_SetSpeed.SetSpeed =...
                    | limitCruiseSpeed(SLA_Sign_Value) - limitOffset;}
                (junction 4571) -> (junction 4570)
                (junction 4572) -> (junction 4571)
                (junction 4573) -> (junction 4572)
                (junction 4570) -> (junction 4574) : %Set new output speed values for display and control
                    | {SET_SetSpdForDispToDrvrVal = PA_DSF_SetSpeed.SetSpeed;
                    | SetSpeedControlOutput(PA_DSF_SetSpeed.SetSpeed)}
              state SPEED_RAMP
                entry:
                fineTuningDone = false;
                state ramp [function]
                  (default) -> (junction 4615)
                  (junction 4615) -> (junction 4616) [order 1] : %Set speed decrease (down button)
                      | [INT_SWSInputData.Button==E_SWSButton.BtnL4Req]
                  (junction 4615) -> (junction 4617) [order 2] : %Increase set speed
                      | {PA_DSF_SetSpeed.SetSpeed =...
                      | limitCruiseSpeed(PA_DSF_SetSpeed.SetSpeed + SetSpeedRamp);}
                  (junction 4616) -> (junction 4619) : %Decrease set speed
                      | {PA_DSF_SetSpeed.SetSpeed =...
                      | limitCruiseSpeed(PA_DSF_SetSpeed.SetSpeed - SetSpeedRamp);}
                  (junction 4617) -> (junction 4618) [order 1] : %SLA valid, SL active and max offset exceeded
                      | [validSLA && PA_DSF_Speed_Limiter_Status==E_CommonStatus.Available &&...
                      | PA_DSF_SetSpeed.SetSpeed - limitCruiseSpeed(SLA_Sign_Value) > limitOffset]
                  (junction 4619) -> (junction 4620) [order 1] : %SLA valid, SL active and max offset exceeded
                      | [validSLA && PA_DSF_Speed_Limiter_Status==E_CommonStatus.Available &&...
                      | PA_DSF_SetSpeed.SetSpeed - limitCruiseSpeed(SLA_Sign_Value) < -limitOffset]
                  (junction 4618) -> (junction 4622) : %Limit to max offset from current speed limit
                      | {PA_DSF_SetSpeed.SetSpeed =...
                      | limitCruiseSpeed(SLA_Sign_Value) + limitOffset;}
                  (junction 4620) -> (junction 4624) : %Limit to max offset from current speed limit
                      | {PA_DSF_SetSpeed.SetSpeed =...
                      | limitCruiseSpeed(SLA_Sign_Value) - limitOffset;}
                  (junction 4617) -> (junction 4621) [order 2]
                  (junction 4619) -> (junction 4623) [order 2]
                  (junction 4622) -> (junction 4621)
                  (junction 4623) -> (junction 4622)
                  (junction 4624) -> (junction 4623)
                  (junction 4621) -> (junction 4625) : %Set new output speed values for display and control
                      | {SET_SetSpdForDispToDrvrVal = PA_DSF_SetSpeed.SetSpeed;
                      | SetSpeedControlOutput(PA_DSF_SetSpeed.SetSpeed)}
                state HOLD_SHORT
                  state RAMP
                    entry: ramp()
                  state IDLE
                  (default) -> SYSTEM_OK.ACTIVE.ACTIVE_A3.SETSPEED_HANDLING.MANUAL_UPDATE.ACTIVE.SPEED_RAMP.HOLD_SHORT.RAMP
                  SYSTEM_OK.ACTIVE.ACTIVE_A3.SETSPEED_HANDLING.MANUAL_UPDATE.ACTIVE.SPEED_RAMP.HOLD_SHORT.RAMP -> SYSTEM_OK.ACTIVE.ACTIVE_A3.SETSPEED_HANDLING.MANUAL_UPDATE.ACTIVE.SPEED_RAMP.HOLD_SHORT.IDLE
                  SYSTEM_OK.ACTIVE.ACTIVE_A3.SETSPEED_HANDLING.MANUAL_UPDATE.ACTIVE.SPEED_RAMP.HOLD_SHORT.IDLE -> SYSTEM_OK.ACTIVE.ACTIVE_A3.SETSPEED_HANDLING.MANUAL_UPDATE.ACTIVE.SPEED_RAMP.HOLD_SHORT.RAMP : after(LCFG_AdjustmentShort, sec)
                state HOLD_LONG_ADJUST_SPEED
                  state IDLE
                  state RAMP
                    entry: ramp()
                  (default) -> SYSTEM_OK.ACTIVE.ACTIVE_A3.SETSPEED_HANDLING.MANUAL_UPDATE.ACTIVE.SPEED_RAMP.HOLD_LONG_ADJUST_SPEED.IDLE
                  SYSTEM_OK.ACTIVE.ACTIVE_A3.SETSPEED_HANDLING.MANUAL_UPDATE.ACTIVE.SPEED_RAMP.HOLD_LONG_ADJUST_SPEED.IDLE -> SYSTEM_OK.ACTIVE.ACTIVE_A3.SETSPEED_HANDLING.MANUAL_UPDATE.ACTIVE.SPEED_RAMP.HOLD_LONG_ADJUST_SPEED.RAMP : after(LCFG_AdjustmentLong, sec)
                  SYSTEM_OK.ACTIVE.ACTIVE_A3.SETSPEED_HANDLING.MANUAL_UPDATE.ACTIVE.SPEED_RAMP.HOLD_LONG_ADJUST_SPEED.RAMP -> SYSTEM_OK.ACTIVE.ACTIVE_A3.SETSPEED_HANDLING.MANUAL_UPDATE.ACTIVE.SPEED_RAMP.HOLD_LONG_ADJUST_SPEED.IDLE
                state FINE_TUNING
                  state FINE_TUNING_DONE
                    entry: fineTuningDone = true
                  state No_RELEASE
                  state RAMP
                  (default) -> SYSTEM_OK.ACTIVE.ACTIVE_A3.SETSPEED_HANDLING.MANUAL_UPDATE.ACTIVE.SPEED_RAMP.FINE_TUNING.RAMP
                  SYSTEM_OK.ACTIVE.ACTIVE_A3.SETSPEED_HANDLING.MANUAL_UPDATE.ACTIVE.SPEED_RAMP.FINE_TUNING.RAMP -> SYSTEM_OK.ACTIVE.ACTIVE_A3.SETSPEED_HANDLING.MANUAL_UPDATE.ACTIVE.SPEED_RAMP.FINE_TUNING.No_RELEASE : [INT_SWSInputData.Event~=E_SWSEvent.Release]
                  SYSTEM_OK.ACTIVE.ACTIVE_A3.SETSPEED_HANDLING.MANUAL_UPDATE.ACTIVE.SPEED_RAMP.FINE_TUNING.No_RELEASE -> SYSTEM_OK.ACTIVE.ACTIVE_A3.SETSPEED_HANDLING.MANUAL_UPDATE.ACTIVE.SPEED_RAMP.FINE_TUNING.FINE_TUNING_DONE [order 2] : after(LCFG_FineTuning, sec)
                  (junction 4653) -> SYSTEM_OK.ACTIVE.ACTIVE_A3.SETSPEED_HANDLING.MANUAL_UPDATE.ACTIVE.SPEED_RAMP.FINE_TUNING.RAMP
                  SYSTEM_OK.ACTIVE.ACTIVE_A3.SETSPEED_HANDLING.MANUAL_UPDATE.ACTIVE.SPEED_RAMP.FINE_TUNING.No_RELEASE -> (junction 4654) [order 1] : [INT_SWSInputData.Event==E_SWSEvent.Release]
                  (junction 4654) -> (junction 4653) : {ramp()}
                (default) -> SYSTEM_OK.ACTIVE.ACTIVE_A3.SETSPEED_HANDLING.MANUAL_UPDATE.ACTIVE.SPEED_RAMP.HOLD_SHORT
                SYSTEM_OK.ACTIVE.ACTIVE_A3.SETSPEED_HANDLING.MANUAL_UPDATE.ACTIVE.SPEED_RAMP.HOLD_SHORT -> SYSTEM_OK.ACTIVE.ACTIVE_A3.SETSPEED_HANDLING.MANUAL_UPDATE.ACTIVE.SPEED_RAMP.HOLD_LONG_ADJUST_SPEED [order 1] : [INT_SWSInputData.Event == E_SWSEvent.HoldLong]
                SYSTEM_OK.ACTIVE.ACTIVE_A3.SETSPEED_HANDLING.MANUAL_UPDATE.ACTIVE.SPEED_RAMP.FINE_TUNING -> SYSTEM_OK.ACTIVE.ACTIVE_A3.SETSPEED_HANDLING.MANUAL_UPDATE.ACTIVE.SPEED_RAMP.HOLD_SHORT : [INT_SWSInputData.Event == E_SWSEvent.HoldShort]
                SYSTEM_OK.ACTIVE.ACTIVE_A3.SETSPEED_HANDLING.MANUAL_UPDATE.ACTIVE.SPEED_RAMP.HOLD_SHORT -> SYSTEM_OK.ACTIVE.ACTIVE_A3.SETSPEED_HANDLING.MANUAL_UPDATE.ACTIVE.SPEED_RAMP.FINE_TUNING [order 2] : [INT_SWSInputData.Event == E_SWSEvent.Release]
                SYSTEM_OK.ACTIVE.ACTIVE_A3.SETSPEED_HANDLING.MANUAL_UPDATE.ACTIVE.SPEED_RAMP.HOLD_LONG_ADJUST_SPEED -> SYSTEM_OK.ACTIVE.ACTIVE_A3.SETSPEED_HANDLING.MANUAL_UPDATE.ACTIVE.SPEED_RAMP.FINE_TUNING : [INT_SWSInputData.Event == E_SWSEvent.Release]
              (default) -> SYSTEM_OK.ACTIVE.ACTIVE_A3.SETSPEED_HANDLING.MANUAL_UPDATE.ACTIVE.REQ_DISABLED
              SYSTEM_OK.ACTIVE.ACTIVE_A3.SETSPEED_HANDLING.MANUAL_UPDATE.ACTIVE.REQ_DISABLED -> SYSTEM_OK.ACTIVE.ACTIVE_A3.SETSPEED_HANDLING.MANUAL_UPDATE.ACTIVE.IDLE : [INT_SWSInputData.Event==E_SWSEvent.Idle &&...
                  | GET_AccSts~=AccSts1.AccSts1_Stop &&...
                  | GET_AccSts~=AccSts1.AccSts1_StopTmp &&...
                  | PA_DSF_Speed_Limit_Adaptation_Value~=...
                  | E_DSF_Value.DSF_Active]
              SYSTEM_OK.ACTIVE.ACTIVE_A3.SETSPEED_HANDLING.MANUAL_UPDATE.ACTIVE.IDLE -> SYSTEM_OK.ACTIVE.ACTIVE_A3.SETSPEED_HANDLING.MANUAL_UPDATE.ACTIVE.REQ_DISABLED [order 1] : %No manual update while stop or SLA
                  | [GET_AccSts==AccSts1.AccSts1_Stop ||...
                  | GET_AccSts==AccSts1.AccSts1_StopTmp ||...
                  | hasChangedTo(PA_DSF_Speed_Limit_Adaptation_Value,...
                  | E_DSF_Value.DSF_Active)]
              SYSTEM_OK.ACTIVE.ACTIVE_A3.SETSPEED_HANDLING.MANUAL_UPDATE.ACTIVE.IDLE -> SYSTEM_OK.ACTIVE.ACTIVE_A3.SETSPEED_HANDLING.MANUAL_UPDATE.ACTIVE.SET_CURRENT_SPEED [order 2] : [(PA_DSF_Adaptive_Cruise_Control_Status==E_CommonStatus.Available) &&...
                  | GET_CrsCtrlOvrdn==OnOff1.OnOff1_On &&...
                  | INT_SWSInputData.Button==E_SWSButton.BtnL5Req &&...
                  | INT_SWSInputData.Event==E_SWSEvent.Push &&...
                  | GET_VehSpdIndcdVal>=PA_DSF_SetSpeed.SetSpeed]
              SYSTEM_OK.ACTIVE.ACTIVE_A3.SETSPEED_HANDLING.MANUAL_UPDATE.ACTIVE.SET_CURRENT_SPEED -> SYSTEM_OK.ACTIVE.ACTIVE_A3.SETSPEED_HANDLING.MANUAL_UPDATE.ACTIVE.IDLE : [INT_SWSInputData.Event == E_SWSEvent.Idle]
              SYSTEM_OK.ACTIVE.ACTIVE_A3.SETSPEED_HANDLING.MANUAL_UPDATE.ACTIVE.IDLE -> SYSTEM_OK.ACTIVE.ACTIVE_A3.SETSPEED_HANDLING.MANUAL_UPDATE.ACTIVE.SPEED_TAP [order 3] : [INT_SWSInputData.Event==E_SWSEvent.Release &&...
                  | (INT_SWSInputData.Button==E_SWSButton.BtnL4Req ||...
                  | INT_SWSInputData.Button==E_SWSButton.BtnL5Req)]
                settings: description=If the up or down button, from the left buttons group, is released.
              SYSTEM_OK.ACTIVE.ACTIVE_A3.SETSPEED_HANDLING.MANUAL_UPDATE.ACTIVE.SPEED_TAP -> SYSTEM_OK.ACTIVE.ACTIVE_A3.SETSPEED_HANDLING.MANUAL_UPDATE.ACTIVE.IDLE : [INT_SWSInputData.Event==E_SWSEvent.Idle]
              SYSTEM_OK.ACTIVE.ACTIVE_A3.SETSPEED_HANDLING.MANUAL_UPDATE.ACTIVE.IDLE -> SYSTEM_OK.ACTIVE.ACTIVE_A3.SETSPEED_HANDLING.MANUAL_UPDATE.ACTIVE.SPEED_RAMP [order 4] : [INT_SWSInputData.Event==E_SWSEvent.HoldShort &&...
                  | (INT_SWSInputData.Button==E_SWSButton.BtnL4Req ||...
                  | INT_SWSInputData.Button==E_SWSButton.BtnL5Req)]
              SYSTEM_OK.ACTIVE.ACTIVE_A3.SETSPEED_HANDLING.MANUAL_UPDATE.ACTIVE.SPEED_RAMP -> SYSTEM_OK.ACTIVE.ACTIVE_A3.SETSPEED_HANDLING.MANUAL_UPDATE.ACTIVE.IDLE : [INT_SWSInputData.Event==E_SWSEvent.Idle && fineTuningDone]
            (default) -> SYSTEM_OK.ACTIVE.ACTIVE_A3.SETSPEED_HANDLING.MANUAL_UPDATE.OFF
            SYSTEM_OK.ACTIVE.ACTIVE_A3.SETSPEED_HANDLING.MANUAL_UPDATE.OFF -> SYSTEM_OK.ACTIVE.ACTIVE_A3.SETSPEED_HANDLING.MANUAL_UPDATE.ACTIVE [order 1] : %Set current speed at SL/ACC activation
                | [hasChangedTo(INT_SL_Event, E_DSF_Event.Activation) ||...
                | (PA_DSF_Speed_Limiter_Value==E_DSF_Value.DSF_Active &&...
                | INT_SL_Event==E_DSF_Event.NoReq) ||...
                | hasChangedTo(INT_ACC_Event, E_DSF_Event.Activation) ||...
                | ((PA_DSF_Adaptive_Cruise_Control_Value==E_DSF_Value.DSF_Active ||...
                | PA_DSF_Adaptive_Cruise_Control_Value==E_DSF_Value.DSF_StopMode) &&...
                | INT_ACC_Event==E_DSF_Event.NoReq)]
                | {PA_DSF_SetSpeed.SetSpeed = limitCruiseSpeed(GET_VehSpdIndcdVal);
                | SET_SetSpdForDispToDrvrVal = PA_DSF_SetSpeed.SetSpeed;
                | SetSpeedControlOutput(PA_DSF_SetSpeed.SetSpeed)}
            SYSTEM_OK.ACTIVE.ACTIVE_A3.SETSPEED_HANDLING.MANUAL_UPDATE.OFF -> SYSTEM_OK.ACTIVE.ACTIVE_A3.SETSPEED_HANDLING.MANUAL_UPDATE.ACTIVE [order 2] : [hasChangedTo(INT_SL_Event, E_DSF_Event.Resume) ||...
                | hasChangedTo(INT_ACC_Event, E_DSF_Event.Resume)]
            SYSTEM_OK.ACTIVE.ACTIVE_A3.SETSPEED_HANDLING.MANUAL_UPDATE.ACTIVE -> SYSTEM_OK.ACTIVE.ACTIVE_A3.SETSPEED_HANDLING.MANUAL_UPDATE.OFF : [PA_DSF_Speed_Limiter_Value==E_DSF_Value.DSF_Standby ||...
                | PA_DSF_Adaptive_Cruise_Control_Value==E_DSF_Value.DSF_Standby]
          state SLA_UPDATE [parallel]
            during: Reset_Offset()
            settings: executionOrder=2
            state REJECTED
              (default) -> (junction 4672)
              (junction 4672) -> (junction 4673) [order 1] : [PA_DSF_SetSpeed.SetSpeed~=0 &&...
                  | PA_DSF_Speed_Limit_Adaptation_Data~=0 &&...
                  | PA_DSF_Speed_Limit_Adaptation_Data~=255 &&...
                  | ctrl_updated]
              (junction 4673) -> (junction 4675) : %Reset control value if updated
                  | {SetSpeedControlOutput(PA_DSF_SetSpeed.SetSpeed);}
              (junction 4672) -> (junction 4674) [order 2]
              (junction 4675) -> (junction 4674)
              (junction 4674) -> (junction 4676)
            state IDLE
            state UPDATE1
              (default) -> (junction 4685)
              (junction 4686) -> (junction 4687) [order 1] : %Update control value immediately at increase
                  | [PA_DSF_Speed_Limit_Adaptation_Data >...
                  | PA_DSF_SetSpeed.SetSpeed]
                  | {SLA_Speed_Change(),...
                  | SetSpeedControlOutput(NewSetSpeed);}
              (junction 4685) -> (junction 4686) [order 1] : [PA_DSF_SetSpeed.SetSpeed~=0 &&...
                  | PA_DSF_Speed_Limit_Adaptation_Data~=0 &&...
                  | PA_DSF_Speed_Limit_Adaptation_Data~=255]
              (junction 4685) -> (junction 4688) [order 2]
              (junction 4686) -> (junction 4689) [order 2] : %Delay control value at decrease
                  | {ctrl_updated = false;}
              (junction 4687) -> (junction 4690) : {ctrl_updated = true;}
              (junction 4689) -> (junction 4688)
              (junction 4690) -> (junction 4689)
              (junction 4688) -> (junction 4691)
            state UPDATE2
              (default) -> (junction 4702)
              (junction 4702) -> (junction 4703) [order 1] : [PA_DSF_SetSpeed.SetSpeed~=0 &&...
                  | PA_DSF_Speed_Limit_Adaptation_Data~=0 &&...
                  | PA_DSF_Speed_Limit_Adaptation_Data~=255]
              (junction 4703) -> (junction 4704) [order 1] : %Update display value at increase
                  | [ctrl_updated]
                  | {PA_DSF_SetSpeed.SetSpeed = NewSetSpeed;
                  | SET_SetSpdForDispToDrvrVal = NewSetSpeed;}
              (junction 4703) -> (junction 4706) [order 2] : %Update both values at decrease
                  | {SLA_Speed_Change()
                  | SetSpeedControlOutput(NewSetSpeed)
                  | PA_DSF_SetSpeed.SetSpeed = NewSetSpeed;
                  | SET_SetSpdForDispToDrvrVal = NewSetSpeed;}
              (junction 4702) -> (junction 4705) [order 2]
              (junction 4704) -> (junction 4707)
              (junction 4706) -> (junction 4705)
              (junction 4707) -> (junction 4706)
              (junction 4705) -> (junction 4708)
            REJECTED -> SYSTEM_OK.ACTIVE.ACTIVE_A3.SETSPEED_HANDLING.SLA_UPDATE.IDLE : [hasChangedTo(PA_DSF_Speed_Limit_Adaptation_Value,...
                | E_DSF_Value.DSF_Standby)]
            UPDATE1 -> REJECTED [order 2] : %Reset values at driver rejection
                | [hasChangedTo(PA_DSF_Speed_Limit_Adaptation_Value,...
                | E_DSF_Value.DSF_Overridden)]
            (default) -> SYSTEM_OK.ACTIVE.ACTIVE_A3.SETSPEED_HANDLING.SLA_UPDATE.IDLE
            SYSTEM_OK.ACTIVE.ACTIVE_A3.SETSPEED_HANDLING.SLA_UPDATE.IDLE -> UPDATE1 : %Initiate SLA at activation
                | [hasChangedTo(PA_DSF_Speed_Limit_Adaptation_Value,...
                | E_DSF_Value.DSF_Active)]
            UPDATE2 -> SYSTEM_OK.ACTIVE.ACTIVE_A3.SETSPEED_HANDLING.SLA_UPDATE.IDLE
            UPDATE1 -> UPDATE2 [order 1] : %Finalize after rejection period
                | [hasChangedTo(PA_DSF_Speed_Limit_Adaptation_Value,...
                | E_DSF_Value.DSF_Standby)]
          state retval = limitCruiseSpeed(val) [function]
            (default) -> (junction 4783)
            (junction 4783) -> (junction 4784) [order 1] : [val < SetSpeedMin]
            (junction 4783) -> (junction 4785) [order 2]
            (junction 4784) -> (junction 4789) : {retval = SetSpeedMin;}
            (junction 4785) -> (junction 4786) [order 1] : [val > SetSpeedMax]
            (junction 4785) -> (junction 4788) [order 2] : {retval = val;}
            (junction 4786) -> (junction 4787) : {retval = SetSpeedMax;}
            (junction 4789) -> (junction 4787)
            (junction 4787) -> (junction 4788)
            (junction 4788) -> (junction 4790)
          state LCFG_Unit_Check [function]
            (default) -> (junction 4862)
            (junction 4862) -> (junction 4863) [order 1] : [GET_SpdUnit==VehSpdIndcdUnit.VehSpdIndcdUnit_Mph]
            (junction 4862) -> (junction 4864) [order 2] : {SetSpeedTap = LCFG_SetSpeedTapKPH;
                | SetSpeedRamp = LCFG_SetSpeedRampKPH;
                | SetSpeedTap2 = LCFG_SetSpeedTap2KPH;}
            (junction 4863) -> (junction 4865) : {SetSpeedTap = LCFG_SetSpeedTapMPH;
                | SetSpeedRamp = LCFG_SetSpeedRampMPH;
                | SetSpeedTap2 = LCFG_SetSpeedTap2MPH;}
            (junction 4865) -> (junction 4864)
            (junction 4864) -> (junction 4866)
          state Reset_Offset [function]
            (default) -> (junction 4750)
            (junction 4750) -> (junction 4751) [order 1] : [PA_DSF_Speed_Limit_Adaptation_Value~=E_DSF_Value.DSF_Active &&...
                | PA_DSF_Speed_Limit_Adaptation_Value~=E_DSF_Value.DSF_Selected &&...
                | PA_DSF_Speed_Limit_Adaptation_Value~=E_DSF_Value.DSF_Standby]
            (junction 4751) -> (junction 4753) : {PA_DSF_SetSpeed.SetSpeed = PA_DSF_SetSpeed.SetSpeed -...
                | PA_DSF_SetSpeed.Offset;
                | PA_DSF_SetSpeed.Offset = 0;}
            (junction 4750) -> (junction 4752) [order 2]
            (junction 4753) -> (junction 4752)
            (junction 4752) -> (junction 4754)
          state unitChange [function]
            (default) -> (junction 4762)
            (junction 4762) -> (junction 4763) [order 1] : [hasChanged(GET_SpdUnit)]
            (junction 4762) -> (junction 4766) [order 2]
            (junction 4763) -> (junction 4764) : {LCFG_Unit_Check();}
            (junction 4764) -> (junction 4765) [order 1] : [GET_SpdUnit==VehSpdIndcdUnit.VehSpdIndcdUnit_Mph]
            (junction 4765) -> (junction 4768) : %Convert from KPH to MPH while making sure we are within
                | % the allowed ranges
                | {PA_DSF_SetSpeed.SetSpeed =...
                | limitCruiseSpeed(floor(64/103*PA_DSF_SetSpeed.SetSpeed));}
            (junction 4764) -> (junction 4767) [order 2] : %Convert from MPH to KPH while making sure we are within
                | % the allowed ranges
                | {PA_DSF_SetSpeed.SetSpeed =...
                | limitCruiseSpeed(floor(103/64*PA_DSF_SetSpeed.SetSpeed));}
            (junction 4767) -> (junction 4766)
            (junction 4768) -> (junction 4767)
            (junction 4766) -> (junction 4769)
          state SetSpeedControlOutput(SetSpeed) [function]
            (default) -> (junction 4875)
            (junction 4875) -> (junction 4876) [order 1] : [PA_SpeedControlFunction_Value==E_OffOn.On]
            (junction 4876) -> (junction 4878) : {SET_SetSpdForCrsCtrlFct =...
                | TrueSpeed(PA_SpeedControlFunction_Data);}
            (junction 4875) -> (junction 4877) [order 2] : {SET_SetSpdForCrsCtrlFct = TrueSpeed(SetSpeed);}
            (junction 4878) -> (junction 4877)
            (junction 4877) -> (junction 4879)
          state ReqSpeed = TrueSpeed(SetSpeed) [function]
            state ConvertedSpeed = RevertConvertedSetSpeed(ConfigMid, ConfigTop, Speed, BreakpointMid, BreakpointTop) [function]
              (default) -> (junction 4829)
              (junction 4829) -> (junction 4830) [order 1] : [Speed==0]
              (junction 4830) -> (junction 4835) : {ConvertedSpeed=0;}
              (junction 4829) -> (junction 4831) [order 2]
              (junction 4831) -> (junction 4832) [order 1] : [Speed<=BreakpointMid]
              (junction 4831) -> (junction 4833) [order 2] : {ConvertedSpeed = Speed-(Speed-BreakpointMid)*(ConfigTop-ConfigMid)/(BreakpointTop-BreakpointMid)-ConfigMid;}
              (junction 4832) -> (junction 4834) : {ConvertedSpeed=Speed-(Speed*ConfigMid/BreakpointMid);}
              (junction 4834) -> (junction 4833)
              (junction 4835) -> (junction 4834)
              (junction 4833) -> (junction 4836)
            state OutputSpeed = ConvertToMeterPerSecond(SpeedToConvert) [function]
              (default) -> (junction 4850)
              (junction 4850) -> (junction 4851) [order 1] : [GET_SpdUnit==VehSpdIndcdUnit.VehSpdIndcdUnit_Mph]
              (junction 4850) -> (junction 4852) [order 2] : {OutputSpeed = SpeedToConvert*10/36;}
              (junction 4851) -> (junction 4853) : {OutputSpeed = SpeedToConvert*515/1152;}
              (junction 4853) -> (junction 4852)
              (junction 4852) -> (junction 4854)
            (default) -> (junction 4804)
            (junction 4804) -> (junction 4805) [order 1] : [cc_param_160==1 || cc_param_160==3 || cc_param_160==5]
            (junction 4804) -> (junction 4806) [order 2]
            (junction 4805) -> (junction 4810) : {ReqSpeed = ConvertToMeterPerSecond(SetSpeed);}
            (junction 4806) -> (junction 4807) [order 1] : [GET_SpdUnit==VehSpdIndcdUnit.VehSpdIndcdUnit_Kmph]
            (junction 4806) -> (junction 4808) [order 2] : %Convert set speed to kph, remove offset and convert to m/s
                | {ReqSpeed = RevertConvertedSetSpeed(LCFG_AddedVehSpdMidOffset,...
                |  LCFG_AddedVehSpdTopOffset, SetSpeed*(103/64),...
                |  LCFG_AddedVehSpdMidOffset + LCFG_ActualVehSpdMid, ...
                |  LCFG_AddedVehSpdTopOffset + LCFG_ActualVehSpdTop)*10/36;}
            (junction 4807) -> (junction 4809) : %Remove offset and convert to m/s
                | {ReqSpeed = RevertConvertedSetSpeed(LCFG_AddedVehSpdMidOffset,...
                |  LCFG_AddedVehSpdTopOffset, SetSpeed,...
                |  LCFG_AddedVehSpdMidOffset + LCFG_ActualVehSpdMid,...
                |  LCFG_AddedVehSpdTopOffset + LCFG_ActualVehSpdTop)*10/36;}
            (junction 4809) -> (junction 4808)
            (junction 4810) -> (junction 4809)
            (junction 4808) -> (junction 4811)
          state SLA_Speed_Change [function]
            (default) -> (junction 4719)
            (junction 4719) -> (junction 4720) [order 1] : %Invalid SLA speed
                | [PA_DSF_Speed_Limit_Adaptation_Data==254]
            (junction 4719) -> (junction 4721) [order 2] : %Set SLA set speed
                | {NewSetSpeed = limitCruiseSpeed(PA_DSF_Speed_Limit_Adaptation_Data);
                | PA_DSF_SetSpeed.Offset = 0;}
            (junction 4720) -> (junction 4722) : {PA_DSF_SetSpeed.Offset = 0;}
            (junction 4722) -> (junction 4721)
            (junction 4721) -> (junction 4723)
      (default) -> (junction 5432)
      (junction 5432) -> ACTIVE_A2 [order 2] : %Argus2
      (junction 5432) -> ACTIVE_A3 [order 1] : %Argus3
          | [cc_param_311==3]
    (default) -> NOT_ACTIVE
    NOT_ACTIVE -> SYSTEM_OK.ACTIVE : [activationCheck()]
    SYSTEM_OK.ACTIVE -> NOT_ACTIVE : [~activationCheck()]
  state SYSTEM_ERROR
    entry:
    PA_DSF_SetSpeed.Status = E_CommonStatus.SystemError;
    PA_DSF_SetSpeed.Value = E_DSF_Value.DSF_Off;
    PA_DSF_SetSpeed.SetSpeed = 0;
    PA_DSF_SetSpeed.Offset = 0;
    SET_SetSpdSts = SetSpdSts1.SetSpdSts1_NoReq;
    SET_SetSpdForCrsCtrlFct = 0;
    SET_SetSpdForDispToDrvrVal = 0;
  (default) -> (junction 3461)
  (junction 3461) -> CARCONFIG_INVALID [order 2]
  (junction 3461) -> (junction 3455) [order 1] : [cc_param_23>1 ||...
      | cc_param_36>1]
  (junction 3455) -> SYSTEM_OK [order 2]
  (junction 3455) -> (junction 3454) [order 1] : [errorCheck()]
  SYSTEM_OK -> SYSTEM_ERROR : [errorCheck()]
  SYSTEM_ERROR -> SYSTEM_OK : [~errorCheck()]
  (junction 3454) -> SYSTEM_ERROR
  data: isError function_output; isActive function_output double; LCFG_SpeedMPH function_input double; retVal function_output double; LCFG_SpeedKPH function_input double; LCFG_MPH function_input double; LCFG_KMPH function_input double; retVal function_output double; ccval function_input double; retVal function_output double; MaxSetSpeed function_input double; retval function_output double; retval function_output; reqsetspeed function_input; reqsetspeed function_input; retval function_output; retVal function_output; offset_max function_output; retval function_output; reqoffset function_input; val function_input double; retval function_output double; manualUpdate local boolean; SetSpeed function_input double; ReqSpeed function_output double; SpeedControlData function_input double; SpeedControlValue function_input Enum: E_OffOn; ConfigMid function_input; ConfigTop function_input; Speed function_input; ConvertedSpeed function_output; BreakpointMid function_input; BreakpointTop function_input; OutPutSpeed function_output; SpeedToConvert function_input; SetSpeed function_input; ReqSpeed function_output; MinSpeedMPH function_input double; retVal function_output double; MinSpeedKPH function_input double; ccval function_input double; retVal function_output double; MaxSpeedMPH function_input double; MaxSpeedKPH function_input double; retVal function_output double; MaxSetSpeed function_input double; retval function_output double; retval function_output; offset_max function_output; retval function_output; reqsetspeed function_input; reqsetspeed function_input; retval function_output; val function_input double; retval function_output double; SetSpeed function_input; ConfigMid function_input; ConfigTop function_input; Speed function_input; ConvertedSpeed function_output; BreakpointMid function_input; BreakpointTop function_input; OutputSpeed function_output; SpeedToConvert function_input; SetSpeed function_input; ReqSpeed function_output; manualUpdate local boolean; PA_DSF_SetSpeed output Bus: PA_StatusAndValueAndDoubleAndDouble; SET_SetSpdSts output Enum: SetSpdSts1; INT_SWSInputData input Bus: SWSInputData; SetSpeedTap local double =5; LCFG_AdjustmentShort parameter; SetSpeedRamp local double =1; fineTuningDone local boolean =false; LCFG_FineTuning parameter; LCFG_AdjustmentLong parameter; SetSpeedMax local double =0; SetSpeedMin local double =0; SET_SetSpdForDispToDrvrVal output double [0..511] =0; GET_VehSpdIndcdVal input double; cc_param_43 parameter; GET_SpdUnit input Enum: VehSpdIndcdUnit; LCFG_SL_SetSpeedMinKPH parameter; LCFG_SL_SetSpeedMinMPH parameter; LCFG_CC_SetSpeedMaxKPH parameter; LCFG_CC_SetSpeedMaxMPH parameter; LCFG_CC_SetSpeedMinKPH parameter; LCFG_CC_SetSpeedMinMPH parameter; LCFG_SetSpeedMaxKPH parameter; LCFG_SetSpeedMaxMPH parameter; LCFG_SetSpeedMinKPH parameter; LCFG_SetSpeedMinMPH parameter; PA_DSF_Speed_Limiter_Status input Enum: E_CommonStatus; PA_DSF_Speed_Limiter_Value input Enum: E_DSF_Value; PA_DSF_Cruise_Control_Status input Enum: E_CommonStatus; PA_DSF_Cruise_Control_Value input Enum: E_DSF_Value; PA_DSF_Adaptive_Cruise_Control_Status input Enum: E_CommonStatus; PA_DSF_Adaptive_Cruise_Control_Value input Enum: E_DSF_Value; SLA_Sign_Value local double =0; LCFG_SL_OffsetReset parameter; GET_SetSpdSelnForAutDrv input Enum: SetSpdSelnForAutDrv1; GET_SpdLimUnit input Enum: SpdUnit1; SLA_Sign_Value_UPDATE local boolean; INT_CC_Event input Enum: E_DSF_Event; INT_SL_Event input Enum: E_DSF_Event; INT_ACC_Event input Enum: E_DSF_Event; LCFG_SetSpeedTapKPH parameter; LCFG_SetSpeedRampMPH parameter; LCFG_SetSpeedTapMPH parameter; LCFG_SetSpeedRampKPH parameter; SET_SetSpdForCrsCtrlFct output double; GET_CrsCtrlOvrdn input Enum: OnOff1; LCFG_SL_MaxOffsetKPH parameter; LCFG_SL_MaxOffsetMPH parameter; PA_DSF_Speed_Limit_Adaptation_Value input Enum: E_DSF_Value; PA_DSF_Speed_Limit_Adaptation_Data input double; cc_param_160 parameter; cc_param_23 parameter; LCFG_SetSpeedTap2KPH parameter; LCFG_SetSpeedTap2MPH parameter; SetSpeedTap2 local double; cc_param_36 parameter; PA_DSF_SL_Warning_Value input Enum: E_OffOn; GET_AdjSpdLimnSts input Enum: AdjSpdLimnSts2; LCFG_AddedVehSpdMidOffset parameter; LCFG_AddedVehSpdTopOffset parameter; LCFG_ActualVehSpdMid parameter; LCFG_ActualVehSpdTop parameter; GET_UsrSeldDrvrSpprtFct input Enum: DrvrSpprtFct; GET_HmiAutnmsStsHmiAutnmsSts input Enum: HmiAutnmsSts1; cc_param_100 parameter; GET_AccSts input Enum: AccSts1; PA_VS_ReducedMaxSpeed_Status input Enum: E_CommonStatus; GET_KeyRstrictdActvSpeedLimit input double; PA_SpeedControlFunction_Status input Enum: E_CommonStatus; PA_SpeedControlFunction_Data input double; PA_SpeedControlFunction_Value input Enum: E_OffOn; updated local; ctrl_updated local; NewSetSpeed local; cc_param_311 parameter; LCFG_SetSpeedMinMPH_A3 parameter; LCFG_SetSpeedMinKPH_A3 parameter
  function retVal = CARCONFIG_MaxSetSpeed(ccval):
    | function retVal = CARCONFIG_MaxSetSpeed(ccval) 
    | switch (ccval)
    |     case 1
    |         retVal=305;
    |         Unit=true; %%true == km per hour
    |     case 2
    |         retVal=100;
    |         Unit=true; %%true == km per hour
    |     case 3
    |         retVal=105;
    |         Unit=true; %%true == km per hour
    |     case 4
    |         retVal=110;
    |         Unit=true; %%true == km per hour
    |     case 5
    |         retVal=115;
    |         Unit=true; %%true == km per hour
    |     case 6
    |         retVal=120;
    |         Unit=true; %%true == km per hour
    |     case 7
    |         retVal=125;
    |         Unit=true; %%true == km per hour
    |     case 8
    |         retVal=130;
    |         Unit=true; %%true == km per hour
    |     case 9
    |         retVal=135;
    |         Unit=true; %%true == km per hour
    |     case 10
    |         retVal=140;
    |         Unit=true; %%true == km per hour
    |     case 11
    |         retVal=145;
    |         Unit=true; %%true == km per hour
    |     case 12
    |         retVal=150;
    |         Unit=true; %%true == km per hour
    |     case 13
    |         retVal=155;
    |         Unit=true; %%true == km per hour
    |     case 14
    |         retVal=160;
    |         Unit=true; %%true == km per hour
    |     case 15
    |         retVal=165;
    |         Unit=true; %%true == km per hour
    |     case 16
    |         retVal=170;
    |         Unit=true; %%true == km per hour
    |     case 17
    |         retVal=175;
    |         Unit=true; %%true == km per hour
    |     case 18
    |         retVal=180;
    |         Unit=true; %%true == km per hour
    |     case 19
    |         retVal=185;
    |         Unit=true; %%true == km per hour
    |     case 20
    |         retVal=190;
    |         Unit=true; %%true == km per hour
    |     case 21
    |         retVal=195;
    |         Unit=true; %%true == km per hour
    |     case 22
    |         retVal=200;
    |         Unit=true; %%true == km per hour
    |     case 23
    |         retVal=205;
    |         Unit=true; %%true == km per hour
    |     case 24
    |         retVal=210;
    |         Unit=true; %%true == km per hour
    |     case 25
    |         retVal=215;
    |         Unit=true; %%true == km per hour
    |     case 26
    |         retVal=220;
    |         Unit=true; %%true == km per hour
    |     case 27
    |         retVal=225;
    |         Unit=true; %%true == km per hour
    |     case 28
    |         retVal=230;
    |         Unit=true; %%true == km per hour
    |     case 29
    |         retVal=235;
    |         Unit=true; %%true == km per hour
    |     case 30
    |         retVal=240;
    |         Unit=true; %%true == km per hour
    |     case 31
    |         retVal=245;
    |         Unit=true; %%true == km per hour
    |     case 32
    |         retVal=250;
    |         Unit=true; %%true == km per hour
    |     case 33
    |         retVal=255;
    |         Unit=true; %%true == km per hour
    |     case 34
    |         retVal=260;
    |         Unit=true; %%true == km per hour
    |     case 35
    |         retVal=265;
    |         Unit=true; %%true == km per hour
    |     case 36
    |         retVal=270;
    |         Unit=true; %%true == km per hour
    |     case 37
    |         retVal=275;
    |         Unit=true; %%true == km per hour
    |     case 38
    |         retVal=280;
    |         Unit=true; %%true == km per hour
    |     case 39
    |         retVal=285;
    |         Unit=true; %%true == km per hour
    |     case 40
    |         retVal=290;
    |         Unit=true; %%true == km per hour
    |     case 41
    |         retVal=295;
    |         Unit=true; %%true == km per hour
    |     case 42
    |         retVal=300;
    |         Unit=true; %%true == km per hour
    |     case 43
    |         retVal=60;
    |         Unit=false; %%true == km per hour
    |     case 44
    |         retVal=65;
    |         Unit=false; %%fasle == miles per hour
    |     case 45
    |         retVal=70;
    |         Unit=false; %%fasle == miles per hour
    |     case 46
    |         retVal=75;
    |         Unit=false; %%fasle == miles per hour
    |     case 47
    |         retVal=80;
    |         Unit=false; %%fasle == miles per hour
    |     case 48
    |         retVal=85;
    |         Unit=false; %%fasle == miles per hour
    |     case 49
    |         retVal=90;
    |         Unit=false; %%fasle == miles per hour
    |     case 50
    |         retVal=95;
    |         Unit=false; %%fasle == miles per hour
    |     case 51
    |         retVal=100;
    |         Unit=false; %%fasle == miles per hour
    |     case 52
    |         retVal=105;
    |         Unit=false; %%fasle == miles per hour
    |     case 53
    |         retVal=110;
    |         Unit=false; %%fasle == miles per hour
    |     case 54
    |         retVal=115;
    |         Unit=false; %%fasle == miles per hour
    |     case 55
    |         retVal=120;
    |         Unit=false; %%fasle == miles per hour
    |     case 56
    |         retVal=125;
    |         Unit=false; %%fasle == miles per hour
    |     case 57
    |         retVal=130;
    |         Unit=false; %%fasle == miles per hour
    |     case 58
    |         retVal=135;
    |         Unit=false; %%fasle == miles per hour
    |     case 59
    |         retVal=140;
    |         Unit=false; %%fasle == miles per hour
    |     case 60
    |         retVal=145;
    |         Unit=false; %%fasle == miles per hour
    |     case 61
    |         retVal=150;
    |         Unit=false; %%fasle == miles per hour
    |     case 62
    |         retVal=155;
    |         Unit=false; %%fasle == miles per hour
    |     case 63
    |         retVal=160;
    |         Unit=false; %%fasle == miles per hour
    |     case 64
    |         retVal=165;
    |         Unit=false; %%fasle == miles per hour
    |     case 65
    |         retVal=170;
    |         Unit=false; %%fasle == miles per hour
    |     case 66
    |         retVal=175;
    |         Unit=false; %%fasle == miles per hour
    |     case 67
    |         retVal=180;
    |         Unit=false; %%fasle == miles per hour
    |     case 68
    |         retVal=185;
    |         Unit=false; %%fasle == miles per hour
    |     case 69
    |         retVal=190;
    |         Unit=false; %%fasle == miles per hour
    |     otherwise
    |         retVal=305;
    |         Unit=true; %%true == km per hour
    | end
    | if (Unit==true) && (GET_SpdUnit==VehSpdIndcdUnit.VehSpdIndcdUnit_Mph)  %%if the cc value states a value in unit kmph but the used unit is mph
    |     retVal=retVal*64/103;
    | elseif (Unit==false) && (GET_SpdUnit==VehSpdIndcdUnit.VehSpdIndcdUnit_Kmph)%%if the cc value states a value in unit mph but the used unit is kmph
    |     retVal=retVal*103/64;
    | end
    | return
  function retVal = CARCONFIG_MaxSetSpeed(ccval):
    | function retVal = CARCONFIG_MaxSetSpeed(ccval) 
    | switch (ccval)
    |     case 1
    |         retVal=305;
    |         Unit=true; %%true == km per hour
    |     case 2
    |         retVal=100;
    |         Unit=true; %%true == km per hour
    |     case 3
    |         retVal=105;
    |         Unit=true; %%true == km per hour
    |     case 4
    |         retVal=110;
    |         Unit=true; %%true == km per hour
    |     case 5
    |         retVal=115;
    |         Unit=true; %%true == km per hour
    |     case 6
    |         retVal=120;
    |         Unit=true; %%true == km per hour
    |     case 7
    |         retVal=125;
    |         Unit=true; %%true == km per hour
    |     case 8
    |         retVal=130;
    |         Unit=true; %%true == km per hour
    |     case 9
    |         retVal=135;
    |         Unit=true; %%true == km per hour
    |     case 10
    |         retVal=140;
    |         Unit=true; %%true == km per hour
    |     case 11
    |         retVal=145;
    |         Unit=true; %%true == km per hour
    |     case 12
    |         retVal=150;
    |         Unit=true; %%true == km per hour
    |     case 13
    |         retVal=155;
    |         Unit=true; %%true == km per hour
    |     case 14
    |         retVal=160;
    |         Unit=true; %%true == km per hour
    |     case 15
    |         retVal=165;
    |         Unit=true; %%true == km per hour
    |     case 16
    |         retVal=170;
    |         Unit=true; %%true == km per hour
    |     case 17
    |         retVal=175;
    |         Unit=true; %%true == km per hour
    |     case 18
    |         retVal=180;
    |         Unit=true; %%true == km per hour
    |     case 19
    |         retVal=185;
    |         Unit=true; %%true == km per hour
    |     case 20
    |         retVal=190;
    |         Unit=true; %%true == km per hour
    |     case 21
    |         retVal=195;
    |         Unit=true; %%true == km per hour
    |     case 22
    |         retVal=200;
    |         Unit=true; %%true == km per hour
    |     case 23
    |         retVal=205;
    |         Unit=true; %%true == km per hour
    |     case 24
    |         retVal=210;
    |         Unit=true; %%true == km per hour
    |     case 25
    |         retVal=215;
    |         Unit=true; %%true == km per hour
    |     case 26
    |         retVal=220;
    |         Unit=true; %%true == km per hour
    |     case 27
    |         retVal=225;
    |         Unit=true; %%true == km per hour
    |     case 28
    |         retVal=230;
    |         Unit=true; %%true == km per hour
    |     case 29
    |         retVal=235;
    |         Unit=true; %%true == km per hour
    |     case 30
    |         retVal=240;
    |         Unit=true; %%true == km per hour
    |     case 31
    |         retVal=245;
    |         Unit=true; %%true == km per hour
    |     case 32
    |         retVal=250;
    |         Unit=true; %%true == km per hour
    |     case 33
    |         retVal=255;
    |         Unit=true; %%true == km per hour
    |     case 34
    |         retVal=260;
    |         Unit=true; %%true == km per hour
    |     case 35
    |         retVal=265;
    |         Unit=true; %%true == km per hour
    |     case 36
    |         retVal=270;
    |         Unit=true; %%true == km per hour
    |     case 37
    |         retVal=275;
    |         Unit=true; %%true == km per hour
    |     case 38
    |         retVal=280;
    |         Unit=true; %%true == km per hour
    |     case 39
    |         retVal=285;
    |         Unit=true; %%true == km per hour
    |     case 40
    |         retVal=290;
    |         Unit=true; %%true == km per hour
    |     case 41
    |         retVal=295;
    |         Unit=true; %%true == km per hour
    |     case 42
    |         retVal=300;
    |         Unit=true; %%true == km per hour
    |     case 43
    |         retVal=60;
    |         Unit=false; %%true == km per hour
    |     case 44
    |         retVal=65;
    |         Unit=false; %%fasle == miles per hour
    |     case 45
    |         retVal=70;
    |         Unit=false; %%fasle == miles per hour
    |     case 46
    |         retVal=75;
    |         Unit=false; %%fasle == miles per hour
    |     case 47
    |         retVal=80;
    |         Unit=false; %%fasle == miles per hour
    |     case 48
    |         retVal=85;
    |         Unit=false; %%fasle == miles per hour
    |     case 49
    |         retVal=90;
    |         Unit=false; %%fasle == miles per hour
    |     case 50
    |         retVal=95;
    |         Unit=false; %%fasle == miles per hour
    |     case 51
    |         retVal=100;
    |         Unit=false; %%fasle == miles per hour
    |     case 52
    |         retVal=105;
    |         Unit=false; %%fasle == miles per hour
    |     case 53
    |         retVal=110;
    |         Unit=false; %%fasle == miles per hour
    |     case 54
    |         retVal=115;
    |         Unit=false; %%fasle == miles per hour
    |     case 55
    |         retVal=120;
    |         Unit=false; %%fasle == miles per hour
    |     case 56
    |         retVal=125;
    |         Unit=false; %%fasle == miles per hour
    |     case 57
    |         retVal=130;
    |         Unit=false; %%fasle == miles per hour
    |     case 58
    |         retVal=135;
    |         Unit=false; %%fasle == miles per hour
    |     case 59
    |         retVal=140;
    |         Unit=false; %%fasle == miles per hour
    |     case 60
    |         retVal=145;
    |         Unit=false; %%fasle == miles per hour
    |     case 61
    |         retVal=150;
    |         Unit=false; %%fasle == miles per hour
    |     case 62
    |         retVal=155;
    |         Unit=false; %%fasle == miles per hour
    |     case 63
    |         retVal=160;
    |         Unit=false; %%fasle == miles per hour
    |     case 64
    |         retVal=165;
    |         Unit=false; %%fasle == miles per hour
    |     case 65
    |         retVal=170;
    |         Unit=false; %%fasle == miles per hour
    |     case 66
    |         retVal=175;
    |         Unit=false; %%fasle == miles per hour
    |     case 67
    |         retVal=180;
    |         Unit=false; %%fasle == miles per hour
    |     case 68
    |         retVal=185;
    |         Unit=false; %%fasle == miles per hour
    |     case 69
    |         retVal=190;
    |         Unit=false; %%fasle == miles per hour
    |     otherwise
    |         retVal=305;
    |         Unit=true; %%true == km per hour
    | end
    | if (Unit==true) && (GET_SpdUnit==VehSpdIndcdUnit.VehSpdIndcdUnit_Mph)  %%if the cc value states a value in unit kmph but the used unit is mph
    |     retVal=retVal*64/103;
    | elseif (Unit==false) && (GET_SpdUnit==VehSpdIndcdUnit.VehSpdIndcdUnit_Kmph)%%if the cc value states a value in unit mph but the used unit is kmph
    |     retVal=retVal*103/64;
    | end
    | return
